simulink model "trim1031"  (R2023b)
settings: Solver=FixedStepAuto  StartTime=0.0  StopTime=200  FixedStep=0.01  RelTol=1e-3
model workspace (MAT data in the model file):
  op_trim1 = opcond.OperatingReport
  op_trim1.Outputs_ = opcond.OutputReport
  op_trim1.Outputs_.yspec_ = [0; 0; 0; 0; 0; 0; 0; 0; 0; 0; 0; 0]
  op_trim1.Outputs_.Block_ = 'trim1031/Output'
  op_trim1.Outputs_.PortWidth_ = 12
  op_trim1.Outputs_.PortNumber_ = NaN
  op_trim1.Outputs_.y_ = [0; 0.0983498986082; 0; -8.56242251282e-06; 0.0451960964113; 8.5624225128e-06; 119.999610613; 2.25043852977e-23; 15.9978397106; 0; 0; -1500.00000422]
  op_trim1.Outputs_.Known_ = [0; 0; 0; 0; 0; 0; 0; 0; 0; 0; 0; 0]
  op_trim1.Outputs_.Min_ = [-Inf; -Inf; -Inf; -Inf; -Inf; -Inf; -Inf; -Inf; -Inf; -Inf; -Inf; -Inf]
  op_trim1.Outputs_.Max_ = [Inf; Inf; Inf; Inf; Inf; Inf; Inf; Inf; Inf; Inf; Inf; Inf]
  op_trim1.TerminationString_ = '成功满足工作点设定。'
  op_trim1.OptimizationOutput_.iterations = 3
  op_trim1.OptimizationOutput_.funcCount = 44
  op_trim1.OptimizationOutput_.lssteplength = 1
  op_trim1.OptimizationOutput_.stepsize = 1.35481389825e-14
  op_trim1.OptimizationOutput_.algorithm = 'active-set'
  op_trim1.OptimizationOutput_.firstorderopt = 0
  op_trim1.OptimizationOutput_.constrviolation = 9.60120871696e-13
  op_trim1.OptimizationOutput_.message = '找到满足约束的局部最小值。
    | 
    | 优化已完成，因为目标函数沿
    | 可行方向在最优性容差值范围内呈现非递减，
    | 并且在约束容差值范围内满足约束。
    | 
    | <停止条件详细信息>
    | 
    | 优化已完成: 一阶最优性测度 0.000000e+00 小于
    | options.OptimalityTolerance = 1.000000e-06，并且最大约束违反值
    | 9.601209e-13 小于 options.ConstraintTolerance = 1.000000e-06。'
  op_trim1.OptimizationOutput_.bestfeasible.x = [0.0983498986082; -8.56242251282e-06; 0.0451960964113; 8.5624225128e-06; 119.999610613; 2.25043852977e-23; 15.9978397106; 0; -1500.00000422; -0.150930640428; 150000; 0; 0]
  op_trim1.OptimizationOutput_.bestfeasible.fval = 0
  op_trim1.OptimizationOutput_.bestfeasible.constrviolation = 9.60120871696e-13
  op_trim1.OptimizationOutput_.bestfeasible.firstorderopt = 0
  op_trim1.OptimizationOutput_.progress = {'<font face="monospaced"; size=3><BR>', '正在优化以求解所有所需的 dx/dt=0、x(k+1)-x(k)=0 和 y=ydes。<BR>', ' <BR>', '(最大误差)模块<BR>', ' ---------------------------------------------------------<BR>', '(4.86343e+00) trim1031/B747 Dynamics动力学参数计算/6DOF Equations of Motion运动学/6DOF (Euler Angles)1/Calculate DCM & Euler Angles/phi theta psi<BR>', '(3.43171e-05) trim1031/B747 Dynamics动力学参数计算/6DOF Equations of Motion运动学/6DOF (Euler Angles)1/Calculate DCM & Euler Angles/phi theta psi<BR>', '(9.60121e-13) trim1031/B747 Dynamics动力学参数计算/6DOF Equations of Motion运动学/6DOF (Euler Angles)1/Calculate DCM & Euler Angles/phi theta psi<BR>', '(9.60121e-13) trim1031/B747 Dynamics动力学参数计算/6DOF Equations of Motion运动学/6DOF (Euler Angles)1/Calculate DCM & Euler Angles/phi theta psi<BR>', ' <BR>', '成功满足工作点设定。<BR>'}
  op_trim1.Model_ = 'trim1031'
  op_trim1.States_(1) = opcond.StateReport
  op_trim1.States_(1).dx_ = [-7.71758340957e-06; 0.0451960964113; 8.60400095293e-06]
  op_trim1.States_(1).Nx_ = 3
  op_trim1.States_(1).Block_ = 'trim1031/B747 Dynamics动力学参数计算/6DOF Equations of Motion运动学/6DOF (Euler Angles)1/Calculate DCM &
    | Euler Angles/phi
    | theta
    | psi'
  op_trim1.States_(1).x_ = [0; 0.0983498986082; 0]
  op_trim1.States_(1).SteadyState_ = [0; 0; 0]
  op_trim1.States_(1).dxMin_ = [-0.3; -0.3; -0.3]
  op_trim1.States_(1).dxMax_ = [0.3; 0.3; 0.3]
  op_trim1.States_(1).Known_ = [1; 0; 1]
  op_trim1.States_(1).Min_ = [-0.5; -0.5; -0.5]
  op_trim1.States_(1).Max_ = [0.5; 0.5; 0.5]
  op_trim1.States_(2) = opcond.StateReport
  op_trim1.States_(2).dx_ = [9.49140044542e-06; 1.90507944892e-15; -1.25297191981e-06]
  op_trim1.States_(2).Nx_ = 3
  op_trim1.States_(2).Block_ = 'trim1031/B747 Dynamics动力学参数计算/6DOF Equations of Motion运动学/6DOF (Euler Angles)1/p,q,r '
  op_trim1.States_(2).x_ = [-8.56242251282e-06; 0.0451960964113; 8.5624225128e-06]
  op_trim1.States_(2).SteadyState_ = [0; 1; 0]
  op_trim1.States_(2).dxMin_ = [-Inf; -Inf; -Inf]
  op_trim1.States_(2).dxMax_ = [Inf; Inf; Inf]
  op_trim1.States_(2).Known_ = [0; 0; 0]
  op_trim1.States_(2).Min_ = [-0.3; -0.3; -0.3]
  op_trim1.States_(2).Max_ = [0.3; 0.3; 0.3]
  op_trim1.States_(3) = opcond.StateReport
  op_trim1.States_(3).dx_ = [0.251459835226; -0.00116446763034; -9.60120871696e-13]
  op_trim1.States_(3).Nx_ = 3
  op_trim1.States_(3).Block_ = 'trim1031/B747 Dynamics动力学参数计算/6DOF Equations of Motion运动学/6DOF (Euler Angles)1/ub,vb,wb'
  op_trim1.States_(3).x_ = [119.999610613; 2.25043852977e-23; 15.9978397106]
  op_trim1.States_(3).SteadyState_ = [0; 0; 1]
  op_trim1.States_(3).dxMin_ = [-Inf; -Inf; -Inf]
  op_trim1.States_(3).dxMax_ = [Inf; Inf; Inf]
  op_trim1.States_(3).Known_ = [0; 0; 0]
  op_trim1.States_(3).Min_ = [0; 0; 0]
  op_trim1.States_(3).Max_ = [Inf; Inf; Inf]
  op_trim1.States_(4) = opcond.StateReport
  op_trim1.States_(4).dx_ = [120.990568654; 2.25043852977e-23; 4.13759827182]
  op_trim1.States_(4).Nx_ = 3
  op_trim1.States_(4).Block_ = 'trim1031/B747 Dynamics动力学参数计算/6DOF Equations of Motion运动学/6DOF (Euler Angles)1/xe,ye,ze'
  op_trim1.States_(4).x_ = [0; 0; -1500.00000422]
  op_trim1.States_(4).SteadyState_ = [0; 1; 0]
  op_trim1.States_(4).dxMin_ = [-Inf; -Inf; -Inf]
  op_trim1.States_(4).dxMax_ = [Inf; Inf; Inf]
  op_trim1.States_(4).Known_ = [0; 1; 0]
  op_trim1.States_(4).Min_ = [-Inf; -Inf; -Inf]
  op_trim1.States_(4).Max_ = [Inf; Inf; 0]
  op_trim1.Inputs_(1) = opcond.InputReport
  op_trim1.Inputs_(1).Block_ = 'trim1031/dE'
  op_trim1.Inputs_(1).PortWidth_ = 1
  op_trim1.Inputs_(1).PortDimensions_ = [1 1]
  op_trim1.Inputs_(1).u_ = -0.150930640428
  op_trim1.Inputs_(1).Known_ = 0
  op_trim1.Inputs_(1).Min_ = -Inf
  op_trim1.Inputs_(1).Max_ = Inf
  op_trim1.Inputs_(2) = opcond.InputReport
  op_trim1.Inputs_(2).Block_ = 'trim1031/dT'
  op_trim1.Inputs_(2).PortWidth_ = 1
  op_trim1.Inputs_(2).PortDimensions_ = [1 1]
  op_trim1.Inputs_(2).u_ = 150000
  op_trim1.Inputs_(2).Known_ = 0
  op_trim1.Inputs_(2).Min_ = 0
  op_trim1.Inputs_(2).Max_ = 240000
  op_trim1.Inputs_(3) = opcond.InputReport
  op_trim1.Inputs_(3).Block_ = 'trim1031/dA'
  op_trim1.Inputs_(3).PortWidth_ = 1
  op_trim1.Inputs_(3).PortDimensions_ = [1 1]
  op_trim1.Inputs_(3).Known_ = 0
  op_trim1.Inputs_(3).Min_ = -Inf
  op_trim1.Inputs_(3).Max_ = Inf
  op_trim1.Inputs_(4) = opcond.InputReport
  op_trim1.Inputs_(4).Block_ = 'trim1031/dR'
  op_trim1.Inputs_(4).PortWidth_ = 1
  op_trim1.Inputs_(4).PortDimensions_ = [1 1]
  op_trim1.Inputs_(4).Known_ = 0
  op_trim1.Inputs_(4).Min_ = -Inf
  op_trim1.Inputs_(4).Max_ = Inf
  op_trim10 = opcond.OperatingReport
  op_trim10.Outputs_ = opcond.OutputReport
  op_trim10.Outputs_.yspec_ = [0; 0; 0; 0; 0; 0; 0; 0; 0; 0; 0; 0]
  op_trim10.Outputs_.Block_ = 'trim1031/Output'
  op_trim10.Outputs_.PortWidth_ = 12
  op_trim10.Outputs_.PortNumber_ = NaN
  op_trim10.Outputs_.y_ = [0; 0.171651347214; 0; -1.07398465823e-08; -0.0379829933296; 1.07398466044e-08; 130.000005709; 9.36786863606e-26; 0.00125401201938; 0; 0; -1499.99999996]
  op_trim10.Outputs_.Known_ = [0; 0; 0; 0; 0; 0; 0; 0; 0; 0; 0; 0]
  op_trim10.Outputs_.Min_ = [-Inf; -Inf; -Inf; -Inf; -Inf; -Inf; -Inf; -Inf; -Inf; -Inf; -Inf; -Inf]
  op_trim10.Outputs_.Max_ = [Inf; Inf; Inf; Inf; Inf; Inf; Inf; Inf; Inf; Inf; Inf; Inf]
  op_trim10.TerminationString_ = '成功满足工作点设定。'
  op_trim10.OptimizationOutput_.iterations = 3
  op_trim10.OptimizationOutput_.funcCount = 44
  op_trim10.OptimizationOutput_.lssteplength = 1
  op_trim10.OptimizationOutput_.stepsize = 3.37664542003e-16
  op_trim10.OptimizationOutput_.algorithm = 'active-set'
  op_trim10.OptimizationOutput_.firstorderopt = 0
  op_trim10.OptimizationOutput_.constrviolation = 2.30926389122e-14
  op_trim10.OptimizationOutput_.message = '找到满足约束的局部最小值。
    | 
    | 优化已完成，因为目标函数沿
    | 可行方向在最优性容差值范围内呈现非递减，
    | 并且在约束容差值范围内满足约束。
    | 
    | <停止条件详细信息>
    | 
    | 优化已完成: 一阶最优性测度 0.000000e+00 小于
    | options.OptimalityTolerance = 1.000000e-06，并且最大约束违反值
    | 2.309264e-14 小于 options.ConstraintTolerance = 1.000000e-06。'
  op_trim10.OptimizationOutput_.bestfeasible.x = [0.171651347214; -1.07398465823e-08; -0.0379829933296; 1.07398466044e-08; 130.000005709; 9.36786863606e-26; 0.00125401201938; 0; -1499.99999996; 0.0383261837012; 192000; 0; 0]
  op_trim10.OptimizationOutput_.bestfeasible.fval = 0
  op_trim10.OptimizationOutput_.bestfeasible.constrviolation = 2.30926389122e-14
  op_trim10.OptimizationOutput_.bestfeasible.firstorderopt = 0
  op_trim10.OptimizationOutput_.progress = {'<font face="monospaced"; size=3><BR>', '正在优化以求解所有所需的 dx/dt=0、x(k+1)-x(k)=0 和 y=ydes。<BR>', ' <BR>', '(最大误差)模块<BR>', ' ---------------------------------------------------------<BR>', '(5.22143e+00) trim1031/B747 Dynamics动力学参数计算/6DOF Equations of Motion运动学/6DOF (Euler Angles)1/p,q,r <BR>', '(1.34354e-05) trim1031/B747 Dynamics动力学参数计算/6DOF Equations of Motion运动学/6DOF (Euler Angles)1/p,q,r <BR>', '(2.30926e-14) trim1031/B747 Dynamics动力学参数计算/6DOF Equations of Motion运动学/6DOF (Euler Angles)1/p,q,r <BR>', '(2.30926e-14) trim1031/B747 Dynamics动力学参数计算/6DOF Equations of Motion运动学/6DOF (Euler Angles)1/p,q,r <BR>', ' <BR>', '成功满足工作点设定。<BR>'}
  op_trim10.Model_ = 'trim1031'
  op_trim10.States_(1) = opcond.StateReport
  op_trim10.States_(1).dx_ = [-8.87801564728e-09; -0.0379829933296; 1.09000330053e-08]
  op_trim10.States_(1).Nx_ = 3
  op_trim10.States_(1).Block_ = 'trim1031/B747 Dynamics动力学参数计算/6DOF Equations of Motion运动学/6DOF (Euler Angles)1/Calculate DCM &
    | Euler Angles/phi
    | theta
    | psi'
  op_trim10.States_(1).x_ = [0; 0.171651347214; 0]
  op_trim10.States_(1).SteadyState_ = [0; 0; 0]
  op_trim10.States_(1).dxMin_ = [-0.3; -0.3; -0.3]
  op_trim10.States_(1).dxMax_ = [0.3; 0.3; 0.3]
  op_trim10.States_(1).Known_ = [1; 0; 1]
  op_trim10.States_(1).Min_ = [-0.5; -0.5; -0.5]
  op_trim10.States_(1).Max_ = [0.5; 0.5; 0.5]
  op_trim10.States_(2) = opcond.StateReport
  op_trim10.States_(2).dx_ = [1.28499584643e-08; -1.21202080755e-16; -2.5916435012e-09]
  op_trim10.States_(2).Nx_ = 3
  op_trim10.States_(2).Block_ = 'trim1031/B747 Dynamics动力学参数计算/6DOF Equations of Motion运动学/6DOF (Euler Angles)1/p,q,r '
  op_trim10.States_(2).x_ = [-1.07398465823e-08; -0.0379829933296; 1.07398466044e-08]
  op_trim10.States_(2).SteadyState_ = [0; 1; 0]
  op_trim10.States_(2).dxMin_ = [-0.03; -0.03; -0.03]
  op_trim10.States_(2).dxMax_ = [0.03; 0.03; 0.03]
  op_trim10.States_(2).Known_ = [0; 0; 0]
  op_trim10.States_(2).Min_ = [-0.3; -0.3; -0.3]
  op_trim10.States_(2).Max_ = [0.3; 0.3; 0.3]
  op_trim10.States_(3) = opcond.StateReport
  op_trim10.States_(3).dx_ = [-1.06099582482; -1.39619358779e-06; -2.30926389122e-14]
  op_trim10.States_(3).Nx_ = 3
  op_trim10.States_(3).Block_ = 'trim1031/B747 Dynamics动力学参数计算/6DOF Equations of Motion运动学/6DOF (Euler Angles)1/ub,vb,wb'
  op_trim10.States_(3).x_ = [130.000005709; 9.36786863606e-26; 0.00125401201938]
  op_trim10.States_(3).SteadyState_ = [0; 0; 1]
  op_trim10.States_(3).dxMin_ = [-Inf; -Inf; -Inf]
  op_trim10.States_(3).dxMax_ = [Inf; Inf; Inf]
  op_trim10.States_(3).Known_ = [0; 0; 0]
  op_trim10.States_(3).Min_ = [0; 0; 0]
  op_trim10.States_(3).Max_ = [Inf; Inf; Inf]
  op_trim10.States_(4) = opcond.StateReport
  op_trim10.States_(4).dx_ = [128.089745597; 9.36786863606e-26; -22.2040212324]
  op_trim10.States_(4).Nx_ = 3
  op_trim10.States_(4).Block_ = 'trim1031/B747 Dynamics动力学参数计算/6DOF Equations of Motion运动学/6DOF (Euler Angles)1/xe,ye,ze'
  op_trim10.States_(4).x_ = [0; 0; -1499.99999996]
  op_trim10.States_(4).SteadyState_ = [0; 1; 0]
  op_trim10.States_(4).dxMin_ = [-Inf; -Inf; -Inf]
  op_trim10.States_(4).dxMax_ = [Inf; Inf; Inf]
  op_trim10.States_(4).Known_ = [0; 1; 0]
  op_trim10.States_(4).Min_ = [-Inf; -Inf; -Inf]
  op_trim10.States_(4).Max_ = [Inf; Inf; 0]
  op_trim10.Inputs_(1) = opcond.InputReport
  op_trim10.Inputs_(1).Block_ = 'trim1031/dE'
  op_trim10.Inputs_(1).PortWidth_ = 1
  op_trim10.Inputs_(1).PortDimensions_ = [1 1]
  op_trim10.Inputs_(1).u_ = 0.0383261837012
  op_trim10.Inputs_(1).Known_ = 0
  op_trim10.Inputs_(1).Min_ = -Inf
  op_trim10.Inputs_(1).Max_ = Inf
  op_trim10.Inputs_(2) = opcond.InputReport
  op_trim10.Inputs_(2).Block_ = 'trim1031/dT'
  op_trim10.Inputs_(2).PortWidth_ = 1
  op_trim10.Inputs_(2).PortDimensions_ = [1 1]
  op_trim10.Inputs_(2).u_ = 192000
  op_trim10.Inputs_(2).Known_ = 0
  op_trim10.Inputs_(2).Min_ = 0
  op_trim10.Inputs_(2).Max_ = 240000
  op_trim10.Inputs_(3) = opcond.InputReport
  op_trim10.Inputs_(3).Block_ = 'trim1031/dA'
  op_trim10.Inputs_(3).PortWidth_ = 1
  op_trim10.Inputs_(3).PortDimensions_ = [1 1]
  op_trim10.Inputs_(3).Known_ = 0
  op_trim10.Inputs_(3).Min_ = -Inf
  op_trim10.Inputs_(3).Max_ = Inf
  op_trim10.Inputs_(4) = opcond.InputReport
  op_trim10.Inputs_(4).Block_ = 'trim1031/dR'
  op_trim10.Inputs_(4).PortWidth_ = 1
  op_trim10.Inputs_(4).PortDimensions_ = [1 1]
  op_trim10.Inputs_(4).Known_ = 0
  op_trim10.Inputs_(4).Min_ = -Inf
  op_trim10.Inputs_(4).Max_ = Inf
  op_trim11 = opcond.OperatingReport
  op_trim11.Outputs_ = opcond.OutputReport
  op_trim11.Outputs_.yspec_ = [0; 0; 0; 0; 0; 0; 0; 0; 0; 0; 0; 0]
  op_trim11.Outputs_.Block_ = 'trim1031/Output'
  op_trim11.Outputs_.PortWidth_ = 12
  op_trim11.Outputs_.PortNumber_ = NaN
  op_trim11.Outputs_.y_ = [0; 0.168996963218; 0; -9.68112442029e-09; 0.0390344222981; 9.6811244158e-09; 129.999918266; 0; 12.9993206248; 0; 0; -1500.0000011]
  op_trim11.Outputs_.Known_ = [0; 0; 0; 0; 0; 0; 0; 0; 0; 0; 0; 0]
  op_trim11.Outputs_.Min_ = [-Inf; -Inf; -Inf; -Inf; -Inf; -Inf; -Inf; -Inf; -Inf; -Inf; -Inf; -Inf]
  op_trim11.Outputs_.Max_ = [Inf; Inf; Inf; Inf; Inf; Inf; Inf; Inf; Inf; Inf; Inf; Inf]
  op_trim11.TerminationString_ = '成功满足工作点设定。'
  op_trim11.OptimizationOutput_.iterations = 4
  op_trim11.OptimizationOutput_.funcCount = 59
  op_trim11.OptimizationOutput_.lssteplength = 1
  op_trim11.OptimizationOutput_.stepsize = 2.96700940297e-15
  op_trim11.OptimizationOutput_.algorithm = 'active-set'
  op_trim11.OptimizationOutput_.firstorderopt = 0
  op_trim11.OptimizationOutput_.constrviolation = 1.7763568394e-14
  op_trim11.OptimizationOutput_.message = '找到满足约束的局部最小值。
    | 
    | 优化已完成，因为目标函数沿
    | 可行方向在最优性容差值范围内呈现非递减，
    | 并且在约束容差值范围内满足约束。
    | 
    | <停止条件详细信息>
    | 
    | 优化已完成: 一阶最优性测度 0.000000e+00 小于
    | options.OptimalityTolerance = 1.000000e-06，并且最大约束违反值
    | 1.776357e-14 小于 options.ConstraintTolerance = 1.000000e-06。'
  op_trim11.OptimizationOutput_.bestfeasible.x = [0.168996963218; -9.68112442029e-09; 0.0390344222981; 9.6811244158e-09; 129.999918266; 0; 12.9993206248; 0; -1500.0000011; -0.0881300190709; 192000; 0; 0]
  op_trim11.OptimizationOutput_.bestfeasible.fval = 0
  op_trim11.OptimizationOutput_.bestfeasible.constrviolation = 1.7763568394e-14
  op_trim11.OptimizationOutput_.bestfeasible.firstorderopt = 0
  op_trim11.OptimizationOutput_.progress = {'<font face="monospaced"; size=3><BR>', '正在优化以求解所有所需的 dx/dt=0、x(k+1)-x(k)=0 和 y=ydes。<BR>', ' <BR>', '(最大误差)模块<BR>', ' ---------------------------------------------------------<BR>', '(4.97990e+00) trim1031/B747 Dynamics动力学参数计算/6DOF Equations of Motion运动学/6DOF (Euler Angles)1/p,q,r <BR>', '(4.08961e-02) trim1031/B747 Dynamics动力学参数计算/6DOF Equations of Motion运动学/6DOF (Euler Angles)1/Calculate DCM & Euler Angles/phi theta psi<BR>', '(1.05395e-06) trim1031/B747 Dynamics动力学参数计算/6DOF Equations of Motion运动学/6DOF (Euler Angles)1/p,q,r <BR>', '(1.77636e-14) trim1031/B747 Dynamics动力学参数计算/6DOF Equations of Motion运动学/6DOF (Euler Angles)1/p,q,r <BR>', '(1.77636e-14) trim1031/B747 Dynamics动力学参数计算/6DOF Equations of Motion运动学/6DOF (Euler Angles)1/p,q,r <BR>', ' <BR>', '成功满足工作点设定。<BR>'}
  op_trim11.Model_ = 'trim1031'
  op_trim11.States_(1) = opcond.StateReport
  op_trim11.States_(1).dx_ = [-8.02928830529e-09; 0.0390344222981; 9.82103520536e-09]
  op_trim11.States_(1).Nx_ = 3
  op_trim11.States_(1).Block_ = 'trim1031/B747 Dynamics动力学参数计算/6DOF Equations of Motion运动学/6DOF (Euler Angles)1/Calculate DCM &
    | Euler Angles/phi
    | theta
    | psi'
  op_trim11.States_(1).x_ = [0; 0.168996963218; 0]
  op_trim11.States_(1).SteadyState_ = [0; 0; 0]
  op_trim11.States_(1).dxMin_ = [-0.3; -0.3; -0.3]
  op_trim11.States_(1).dxMax_ = [0.3; 0.3; 0.3]
  op_trim11.States_(1).Known_ = [1; 0; 1]
  op_trim11.States_(1).Min_ = [-0.5; -0.5; -0.5]
  op_trim11.States_(1).Max_ = [0.5; 0.5; 0.5]
  op_trim11.States_(2) = opcond.StateReport
  op_trim11.States_(2).dx_ = [1.15109176436e-08; -0.03; -1.70079708465e-09]
  op_trim11.States_(2).Nx_ = 3
  op_trim11.States_(2).Block_ = 'trim1031/B747 Dynamics动力学参数计算/6DOF Equations of Motion运动学/6DOF (Euler Angles)1/p,q,r '
  op_trim11.States_(2).x_ = [-9.68112442029e-09; 0.0390344222981; 9.6811244158e-09]
  op_trim11.States_(2).SteadyState_ = [0; 0; 0]
  op_trim11.States_(2).dxMin_ = [-0.03; -0.03; -0.03]
  op_trim11.States_(2).dxMax_ = [0.03; 0.03; 0.03]
  op_trim11.States_(2).Known_ = [0; 0; 0]
  op_trim11.States_(2).Min_ = [-0.3; -0.3; -0.3]
  op_trim11.States_(2).Max_ = [0.3; 0.3; 0.3]
  op_trim11.States_(3) = opcond.StateReport
  op_trim11.States_(3).dx_ = [-0.537845537105; -1.38439342313e-06; -1.7763568394e-14]
  op_trim11.States_(3).Nx_ = 3
  op_trim11.States_(3).Block_ = 'trim1031/B747 Dynamics动力学参数计算/6DOF Equations of Motion运动学/6DOF (Euler Angles)1/ub,vb,wb'
  op_trim11.States_(3).x_ = [129.999918266; 0; 12.9993206248]
  op_trim11.States_(3).SteadyState_ = [0; 0; 1]
  op_trim11.States_(3).dxMin_ = [-Inf; -Inf; -Inf]
  op_trim11.States_(3).dxMax_ = [Inf; Inf; Inf]
  op_trim11.States_(3).Known_ = [0; 0; 0]
  op_trim11.States_(3).Min_ = [0; 0; 0]
  op_trim11.States_(3).Max_ = [Inf; Inf; Inf]
  op_trim11.States_(4) = opcond.StateReport
  op_trim11.States_(4).dx_ = [130.334338824; 0; -9.05103360207]
  op_trim11.States_(4).Nx_ = 3
  op_trim11.States_(4).Block_ = 'trim1031/B747 Dynamics动力学参数计算/6DOF Equations of Motion运动学/6DOF (Euler Angles)1/xe,ye,ze'
  op_trim11.States_(4).x_ = [0; 0; -1500.0000011]
  op_trim11.States_(4).SteadyState_ = [0; 1; 0]
  op_trim11.States_(4).dxMin_ = [-Inf; -Inf; -Inf]
  op_trim11.States_(4).dxMax_ = [Inf; Inf; Inf]
  op_trim11.States_(4).Known_ = [0; 1; 0]
  op_trim11.States_(4).Min_ = [-Inf; -Inf; -Inf]
  op_trim11.States_(4).Max_ = [Inf; Inf; 0]
  op_trim11.Inputs_(1) = opcond.InputReport
  op_trim11.Inputs_(1).Block_ = 'trim1031/dE'
  op_trim11.Inputs_(1).PortWidth_ = 1
  op_trim11.Inputs_(1).PortDimensions_ = [1 1]
  op_trim11.Inputs_(1).u_ = -0.0881300190709
  op_trim11.Inputs_(1).Known_ = 0
  op_trim11.Inputs_(1).Min_ = -Inf
  op_trim11.Inputs_(1).Max_ = Inf
  op_trim11.Inputs_(2) = opcond.InputReport
  op_trim11.Inputs_(2).Block_ = 'trim1031/dT'
  op_trim11.Inputs_(2).PortWidth_ = 1
  op_trim11.Inputs_(2).PortDimensions_ = [1 1]
  op_trim11.Inputs_(2).u_ = 192000
  op_trim11.Inputs_(2).Known_ = 0
  op_trim11.Inputs_(2).Min_ = 0
  op_trim11.Inputs_(2).Max_ = 240000
  op_trim11.Inputs_(3) = opcond.InputReport
  op_trim11.Inputs_(3).Block_ = 'trim1031/dA'
  op_trim11.Inputs_(3).PortWidth_ = 1
  op_trim11.Inputs_(3).PortDimensions_ = [1 1]
  op_trim11.Inputs_(3).Known_ = 0
  op_trim11.Inputs_(3).Min_ = -Inf
  op_trim11.Inputs_(3).Max_ = Inf
  op_trim11.Inputs_(4) = opcond.InputReport
  op_trim11.Inputs_(4).Block_ = 'trim1031/dR'
  op_trim11.Inputs_(4).PortWidth_ = 1
  op_trim11.Inputs_(4).PortDimensions_ = [1 1]
  op_trim11.Inputs_(4).Known_ = 0
  op_trim11.Inputs_(4).Min_ = -Inf
  op_trim11.Inputs_(4).Max_ = Inf
  op_trim12 = opcond.OperatingReport
  op_trim12.Outputs_ = opcond.OutputReport
  op_trim12.Outputs_.yspec_ = [0; 0; 0; 0; 0; 0; 0; 0; 0; 0; 0; 0]
  op_trim12.Outputs_.Block_ = 'trim1031/Output'
  op_trim12.Outputs_.PortWidth_ = 12
  op_trim12.Outputs_.PortNumber_ = NaN
  op_trim12.Outputs_.y_ = [0; 0.167988525312; 0; 1.78845872578e-25; -0.00250420987712; 1e-05; 129.999998768; -2.5381879176e-33; 13.0000321666; 0; 0; -1499.99999999]
  op_trim12.Outputs_.Known_ = [0; 0; 0; 0; 0; 0; 0; 0; 0; 0; 0; 0]
  op_trim12.Outputs_.Min_ = [-Inf; -Inf; -Inf; -Inf; -Inf; -Inf; -Inf; -Inf; -Inf; -Inf; -Inf; -Inf]
  op_trim12.Outputs_.Max_ = [Inf; Inf; Inf; Inf; Inf; Inf; Inf; Inf; Inf; Inf; Inf; Inf]
  op_trim12.TerminationString_ = '成功满足工作点设定。'
  op_trim12.OptimizationOutput_.iterations = 2
  op_trim12.OptimizationOutput_.funcCount = 44
  op_trim12.OptimizationOutput_.lssteplength = 1
  op_trim12.OptimizationOutput_.stepsize = 2.2121751606e-07
  op_trim12.OptimizationOutput_.algorithm = 'active-set'
  op_trim12.OptimizationOutput_.firstorderopt = 2.36442055551e-11
  op_trim12.OptimizationOutput_.constrviolation = 1.41622824579e-14
  op_trim12.OptimizationOutput_.message = '找到满足约束的局部最小值。
    | 
    | 优化已完成，因为目标函数沿
    | 可行方向在最优性容差值范围内呈现非递减，
    | 并且在约束容差值范围内满足约束。
    | 
    | <停止条件详细信息>
    | 
    | 优化已完成: 一阶最优性测度 2.364421e-11 小于
    | options.OptimalityTolerance = 1.000000e-06，并且最大约束违反值
    | 1.416228e-14 小于 options.ConstraintTolerance = 1.000000e-06。'
  op_trim12.OptimizationOutput_.bestfeasible.x = [0.167988525312; 1.78845872578e-25; -0.00250420987712; 1e-05; 129.999998768; -2.5381879176e-33; 13.0000321666; 0; -1499.99999999; -0.0498466910775; 192000; 0; 0]
  op_trim12.OptimizationOutput_.bestfeasible.fval = 0
  op_trim12.OptimizationOutput_.bestfeasible.constrviolation = 1.41622824579e-14
  op_trim12.OptimizationOutput_.bestfeasible.firstorderopt = 2.36442055551e-11
  op_trim12.OptimizationOutput_.progress = {'<font face="monospaced"; size=3><BR>', '正在优化以求解所有所需的 dx/dt=0、x(k+1)-x(k)=0 和 y=ydes。<BR>', ' <BR>', '(最大误差)模块<BR>', ' ---------------------------------------------------------<BR>', '(4.96933e-02) trim1031/B747 Dynamics动力学参数计算/6DOF Equations of Motion运动学/6DOF (Euler Angles)1/p,q,r <BR>', '(3.41872e-06) trim1031/B747 Dynamics动力学参数计算/6DOF Equations of Motion运动学/6DOF (Euler Angles)1/p,q,r <BR>', '(1.41623e-14) trim1031/B747 Dynamics动力学参数计算/6DOF Equations of Motion运动学/6DOF (Euler Angles)1/p,q,r <BR>', '(1.41623e-14) trim1031/B747 Dynamics动力学参数计算/6DOF Equations of Motion运动学/6DOF (Euler Angles)1/p,q,r <BR>', ' <BR>', '成功满足工作点设定。<BR>'}
  op_trim12.Model_ = 'trim1031'
  op_trim12.States_(1) = opcond.StateReport
  op_trim12.States_(1).dx_ = [1.69586789196e-06; -0.00250420987712; 1.01427791018e-05]
  op_trim12.States_(1).Nx_ = 3
  op_trim12.States_(1).Block_ = 'trim1031/B747 Dynamics动力学参数计算/6DOF Equations of Motion运动学/6DOF (Euler Angles)1/Calculate DCM &
    | Euler Angles/phi
    | theta
    | psi'
  op_trim12.States_(1).x_ = [0; 0.167988525312; 0]
  op_trim12.States_(1).SteadyState_ = [0; 0; 0]
  op_trim12.States_(1).dxMin_ = [-0.3; -0.3; -0.3]
  op_trim12.States_(1).dxMax_ = [0.3; 0.3; 0.3]
  op_trim12.States_(1).Known_ = [1; 0; 1]
  op_trim12.States_(1).Min_ = [-0.5; -0.5; -0.5]
  op_trim12.States_(1).Max_ = [0.5; 0.5; 0.5]
  op_trim12.States_(2) = opcond.StateReport
  op_trim12.States_(2).dx_ = [3.92855222752e-06; -0.0262934164576; -2.41695804279e-06]
  op_trim12.States_(2).Nx_ = 3
  op_trim12.States_(2).Block_ = 'trim1031/B747 Dynamics动力学参数计算/6DOF Equations of Motion运动学/6DOF (Euler Angles)1/p,q,r '
  op_trim12.States_(2).x_ = [1.78845872578e-25; -0.00250420987712; 1e-05]
  op_trim12.States_(2).SteadyState_ = [0; 0; 0]
  op_trim12.States_(2).dxMin_ = [-0.03; -0.03; -0.03]
  op_trim12.States_(2).dxMax_ = [0.03; 0.03; 0.03]
  op_trim12.States_(2).Known_ = [0; 0; 0]
  op_trim12.States_(2).Min_ = [-0.3; -0.3; -0.3]
  op_trim12.States_(2).Max_ = [0.3; 0.3; 0.3]
  op_trim12.States_(3) = opcond.StateReport
  op_trim12.States_(3).dx_ = [1.41622824579e-14; -0.00129999998768; -5.27904040513]
  op_trim12.States_(3).Nx_ = 3
  op_trim12.States_(3).Block_ = 'trim1031/B747 Dynamics动力学参数计算/6DOF Equations of Motion运动学/6DOF (Euler Angles)1/ub,vb,wb'
  op_trim12.States_(3).x_ = [129.999998768; -2.5381879176e-33; 13.0000321666]
  op_trim12.States_(3).SteadyState_ = [1; 0; 0]
  op_trim12.States_(3).dxMin_ = [-Inf; -Inf; -Inf]
  op_trim12.States_(3).dxMax_ = [Inf; Inf; Inf]
  op_trim12.States_(3).Known_ = [0; 0; 0]
  op_trim12.States_(3).Min_ = [0; 0; 0]
  op_trim12.States_(3).Max_ = [Inf; Inf; Inf]
  op_trim12.States_(4) = opcond.StateReport
  op_trim12.States_(4).dx_ = [130.343598294; -2.5381879176e-33; -8.9189068687]
  op_trim12.States_(4).Nx_ = 3
  op_trim12.States_(4).Block_ = 'trim1031/B747 Dynamics动力学参数计算/6DOF Equations of Motion运动学/6DOF (Euler Angles)1/xe,ye,ze'
  op_trim12.States_(4).x_ = [0; 0; -1499.99999999]
  op_trim12.States_(4).SteadyState_ = [0; 1; 0]
  op_trim12.States_(4).dxMin_ = [-Inf; -Inf; -Inf]
  op_trim12.States_(4).dxMax_ = [Inf; Inf; Inf]
  op_trim12.States_(4).Known_ = [0; 1; 0]
  op_trim12.States_(4).Min_ = [-Inf; -Inf; -Inf]
  op_trim12.States_(4).Max_ = [Inf; Inf; 0]
  op_trim12.Inputs_(1) = opcond.InputReport
  op_trim12.Inputs_(1).Block_ = 'trim1031/dE'
  op_trim12.Inputs_(1).PortWidth_ = 1
  op_trim12.Inputs_(1).PortDimensions_ = [1 1]
  op_trim12.Inputs_(1).u_ = -0.0498466910775
  op_trim12.Inputs_(1).Known_ = 0
  op_trim12.Inputs_(1).Min_ = -Inf
  op_trim12.Inputs_(1).Max_ = Inf
  op_trim12.Inputs_(2) = opcond.InputReport
  op_trim12.Inputs_(2).Block_ = 'trim1031/dT'
  op_trim12.Inputs_(2).PortWidth_ = 1
  op_trim12.Inputs_(2).PortDimensions_ = [1 1]
  op_trim12.Inputs_(2).u_ = 192000
  op_trim12.Inputs_(2).Known_ = 0
  op_trim12.Inputs_(2).Min_ = 0
  op_trim12.Inputs_(2).Max_ = 240000
  op_trim12.Inputs_(3) = opcond.InputReport
  op_trim12.Inputs_(3).Block_ = 'trim1031/dA'
  op_trim12.Inputs_(3).PortWidth_ = 1
  op_trim12.Inputs_(3).PortDimensions_ = [1 1]
  op_trim12.Inputs_(3).Known_ = 0
  op_trim12.Inputs_(3).Min_ = -Inf
  op_trim12.Inputs_(3).Max_ = Inf
  op_trim12.Inputs_(4) = opcond.InputReport
  op_trim12.Inputs_(4).Block_ = 'trim1031/dR'
  op_trim12.Inputs_(4).PortWidth_ = 1
  op_trim12.Inputs_(4).PortDimensions_ = [1 1]
  op_trim12.Inputs_(4).Known_ = 0
  op_trim12.Inputs_(4).Min_ = -Inf
  op_trim12.Inputs_(4).Max_ = Inf
  op_trim13 = opcond.OperatingReport
  op_trim13.Outputs_ = opcond.OutputReport
  op_trim13.Outputs_.yspec_ = [0; 0; 0; 0; 0; 0; 0; 0; 0; 0; 0; 0]
  op_trim13.Outputs_.Block_ = 'trim1031/Output'
  op_trim13.Outputs_.PortWidth_ = 12
  op_trim13.Outputs_.PortNumber_ = NaN
  op_trim13.Outputs_.y_ = [0.0001; 0.1; 6.28308530718; -0.000179538158685; -0.00751789694975; -1.41195963211e-05; 121.02593479; 0.0127716364451; 6.63287181793; -2.82407339315e-17; 0; -1499.99553412]
  op_trim13.Outputs_.Known_ = [0; 0; 0; 0; 0; 0; 0; 0; 0; 0; 0; 0]
  op_trim13.Outputs_.Min_ = [-Inf; -Inf; -Inf; -Inf; -Inf; -Inf; -Inf; -Inf; -Inf; -Inf; -Inf; -Inf]
  op_trim13.Outputs_.Max_ = [Inf; Inf; Inf; Inf; Inf; Inf; Inf; Inf; Inf; Inf; Inf; Inf]
  op_trim13.TerminationString_ = '成功满足工作点设定。'
  op_trim13.OptimizationOutput_.iterations = 4
  op_trim13.OptimizationOutput_.funcCount = 55
  op_trim13.OptimizationOutput_.lssteplength = 1
  op_trim13.OptimizationOutput_.stepsize = 1.07319719222e-09
  op_trim13.OptimizationOutput_.algorithm = 'active-set'
  op_trim13.OptimizationOutput_.firstorderopt = 0
  op_trim13.OptimizationOutput_.constrviolation = 2.33658647986e-11
  op_trim13.OptimizationOutput_.message = '找到满足约束的局部最小值。
    | 
    | 优化已完成，因为目标函数沿
    | 可行方向在最优性容差值范围内呈现非递减，
    | 并且在约束容差值范围内满足约束。
    | 
    | <停止条件详细信息>
    | 
    | 优化已完成: 一阶最优性测度 0.000000e+00 小于
    | options.OptimalityTolerance = 1.000000e-06，并且最大约束违反值
    | 2.336586e-11 小于 options.ConstraintTolerance = 1.000000e-06。'
  op_trim13.OptimizationOutput_.bestfeasible.x = [-0.000179538158685; -0.00751789694975; -1.41195963211e-05; 121.02593479; 0.0127716364451; 6.63287181793; -2.82407339315e-17; -1499.99553412; -0.0124968353108; 191999.999642; -2.78444784735e-05; 0.00018916555193]
  op_trim13.OptimizationOutput_.bestfeasible.fval = 0
  op_trim13.OptimizationOutput_.bestfeasible.constrviolation = 2.33658647986e-11
  op_trim13.OptimizationOutput_.bestfeasible.firstorderopt = 0
  op_trim13.OptimizationOutput_.progress = {'<font face="monospaced"; size=3><BR>', '正在优化以求解所有所需的 dx/dt=0、x(k+1)-x(k)=0 和 y=ydes。<BR>', ' <BR>', '(最大误差)模块<BR>', ' ---------------------------------------------------------<BR>', '(1.84926e-01) trim1031/B747 Dynamics动力学参数计算/6DOF Equations of Motion运动学/6DOF (Euler Angles)1/xe,ye,ze<BR>', '(6.48574e-03) trim1031/B747 Dynamics动力学参数计算/6DOF Equations of Motion运动学/6DOF (Euler Angles)1/xe,ye,ze<BR>', '(9.24667e-06) trim1031/B747 Dynamics动力学参数计算/6DOF Equations of Motion运动学/6DOF (Euler Angles)1/xe,ye,ze<BR>', '(2.33659e-11) trim1031/B747 Dynamics动力学参数计算/6DOF Equations of Motion运动学/6DOF (Euler Angles)1/p,q,r <BR>', '(2.33659e-11) trim1031/B747 Dynamics动力学参数计算/6DOF Equations of Motion运动学/6DOF (Euler Angles)1/p,q,r <BR>', ' <BR>', '成功满足工作点设定。<BR>'}
  op_trim13.Model_ = 'trim1031'
  op_trim13.States_(1) = opcond.StateReport
  op_trim13.States_(1).dx_ = [-0.000181030274317; -0.0075178955002; -1.49460539596e-05]
  op_trim13.States_(1).Nx_ = 3
  op_trim13.States_(1).Block_ = 'trim1031/B747 Dynamics动力学参数计算/6DOF Equations of Motion运动学/6DOF (Euler Angles)1/Calculate DCM &
    | Euler Angles/phi
    | theta
    | psi'
  op_trim13.States_(1).x_ = [0.0001; 0.1; -0.0001]
  op_trim13.States_(1).SteadyState_ = [0; 0; 0]
  op_trim13.States_(1).dxMin_ = [-Inf; -0.2; -Inf]
  op_trim13.States_(1).dxMax_ = [Inf; 0.2; Inf]
  op_trim13.States_(1).Known_ = [1; 1; 1]
  op_trim13.States_(1).Min_ = [-Inf; -0.51; -Inf]
  op_trim13.States_(1).Max_ = [Inf; 0.51; Inf]
  op_trim13.States_(2) = opcond.StateReport
  op_trim13.States_(2).dx_ = [-3.34973655326e-15; -0.0200000000005; 5.67519754943e-15]
  op_trim13.States_(2).Nx_ = 3
  op_trim13.States_(2).Block_ = 'trim1031/B747 Dynamics动力学参数计算/6DOF Equations of Motion运动学/6DOF (Euler Angles)1/p,q,r '
  op_trim13.States_(2).x_ = [-0.000179538158685; -0.00751789694975; -1.41195963211e-05]
  op_trim13.States_(2).SteadyState_ = [1; 0; 1]
  op_trim13.States_(2).dxMin_ = [-Inf; -0.02; -Inf]
  op_trim13.States_(2).dxMax_ = [Inf; 0.02; Inf]
  op_trim13.States_(2).Known_ = [0; 0; 0]
  op_trim13.States_(2).Min_ = [-Inf; -0.2; -Inf]
  op_trim13.States_(2).Max_ = [Inf; 0.2; Inf]
  op_trim13.States_(3) = opcond.StateReport
  op_trim13.States_(3).dx_ = [1.83950285559e-11; -1.552358719e-12; -2.33658647986e-11]
  op_trim13.States_(3).Nx_ = 3
  op_trim13.States_(3).Block_ = 'trim1031/B747 Dynamics动力学参数计算/6DOF Equations of Motion运动学/6DOF (Euler Angles)1/ub,vb,wb'
  op_trim13.States_(3).x_ = [121.02593479; 0.0127716364451; 6.63287181793]
  op_trim13.States_(3).SteadyState_ = [1; 1; 1]
  op_trim13.States_(3).dxMin_ = [-Inf; -Inf; -Inf]
  op_trim13.States_(3).dxMax_ = [Inf; Inf; Inf]
  op_trim13.States_(3).Known_ = [0; 0; 0]
  op_trim13.States_(3).Min_ = [0; 0; 0]
  op_trim13.States_(3).Max_ = [Inf; Inf; Inf]
  op_trim13.States_(4) = opcond.StateReport
  op_trim13.States_(4).dx_ = [121.083492208; 1.99493199737e-17; -5.48269624853]
  op_trim13.States_(4).Nx_ = 3
  op_trim13.States_(4).Block_ = 'trim1031/B747 Dynamics动力学参数计算/6DOF Equations of Motion运动学/6DOF (Euler Angles)1/xe,ye,ze'
  op_trim13.States_(4).x_ = [-2.82407339315e-17; 0; -1499.99553412]
  op_trim13.States_(4).SteadyState_ = [0; 1; 0]
  op_trim13.States_(4).dxMin_ = [-Inf; -Inf; -100]
  op_trim13.States_(4).dxMax_ = [Inf; Inf; 100]
  op_trim13.States_(4).Known_ = [0; 1; 0]
  op_trim13.States_(4).Min_ = [0; -Inf; -Inf]
  op_trim13.States_(4).Max_ = [Inf; Inf; 0]
  op_trim13.Inputs_(1) = opcond.InputReport
  op_trim13.Inputs_(1).Block_ = 'trim1031/dE'
  op_trim13.Inputs_(1).PortWidth_ = 1
  op_trim13.Inputs_(1).PortDimensions_ = [1 1]
  op_trim13.Inputs_(1).u_ = -0.0124968353108
  op_trim13.Inputs_(1).Known_ = 0
  op_trim13.Inputs_(1).Min_ = -Inf
  op_trim13.Inputs_(1).Max_ = Inf
  op_trim13.Inputs_(2) = opcond.InputReport
  op_trim13.Inputs_(2).Block_ = 'trim1031/dT'
  op_trim13.Inputs_(2).PortWidth_ = 1
  op_trim13.Inputs_(2).PortDimensions_ = [1 1]
  op_trim13.Inputs_(2).u_ = 191999.999642
  op_trim13.Inputs_(2).Known_ = 0
  op_trim13.Inputs_(2).Min_ = -Inf
  op_trim13.Inputs_(2).Max_ = Inf
  op_trim13.Inputs_(3) = opcond.InputReport
  op_trim13.Inputs_(3).Block_ = 'trim1031/dA'
  op_trim13.Inputs_(3).PortWidth_ = 1
  op_trim13.Inputs_(3).PortDimensions_ = [1 1]
  op_trim13.Inputs_(3).u_ = -2.78444784735e-05
  op_trim13.Inputs_(3).Known_ = 0
  op_trim13.Inputs_(3).Min_ = -0.001
  op_trim13.Inputs_(3).Max_ = 0.001
  op_trim13.Inputs_(4) = opcond.InputReport
  op_trim13.Inputs_(4).Block_ = 'trim1031/dR'
  op_trim13.Inputs_(4).PortWidth_ = 1
  op_trim13.Inputs_(4).PortDimensions_ = [1 1]
  op_trim13.Inputs_(4).u_ = 0.00018916555193
  op_trim13.Inputs_(4).Known_ = 0
  op_trim13.Inputs_(4).Min_ = -0.001
  op_trim13.Inputs_(4).Max_ = 0.001
  op_trim14 = opcond.OperatingReport
  op_trim14.Outputs_ = opcond.OutputReport
  op_trim14.Outputs_.yspec_ = [0; 0; 0; 0; 0; 0; 0; 0; 0; 0; 0; 0]
  op_trim14.Outputs_.Block_ = 'trim1031/Output'
  op_trim14.Outputs_.PortWidth_ = 12
  op_trim14.Outputs_.PortNumber_ = NaN
  op_trim14.Outputs_.y_ = [0.0001; 0.117526200284; 6.28308530718; -0.000189020429197; 0.0101067920949; -2.02135516275e-05; 120.000004191; 0.0130344316639; 9.99959180984; 0; 0; -1500.0000002]
  op_trim14.Outputs_.Known_ = [0; 0; 0; 0; 0; 0; 0; 0; 0; 0; 0; 0]
  op_trim14.Outputs_.Min_ = [-Inf; -Inf; -Inf; -Inf; -Inf; -Inf; -Inf; -Inf; -Inf; -Inf; -Inf; -Inf]
  op_trim14.Outputs_.Max_ = [Inf; Inf; Inf; Inf; Inf; Inf; Inf; Inf; Inf; Inf; Inf; Inf]
  op_trim14.TerminationString_ = '成功满足工作点设定。'
  op_trim14.OptimizationOutput_.iterations = 3
  op_trim14.OptimizationOutput_.funcCount = 44
  op_trim14.OptimizationOutput_.lssteplength = 1
  op_trim14.OptimizationOutput_.stepsize = 6.32859168734e-11
  op_trim14.OptimizationOutput_.algorithm = 'active-set'
  op_trim14.OptimizationOutput_.firstorderopt = 0
  op_trim14.OptimizationOutput_.constrviolation = 7.22555348887e-11
  op_trim14.OptimizationOutput_.message = '找到满足约束的局部最小值。
    | 
    | 优化已完成，因为目标函数沿
    | 可行方向在最优性容差值范围内呈现非递减，
    | 并且在约束容差值范围内满足约束。
    | 
    | <停止条件详细信息>
    | 
    | 优化已完成: 一阶最优性测度 0.000000e+00 小于
    | options.OptimalityTolerance = 1.000000e-06，并且最大约束违反值
    | 7.225553e-11 小于 options.ConstraintTolerance = 1.000000e-06。'
  op_trim14.OptimizationOutput_.bestfeasible.x = [0.117526200284; -0.000189020429197; 0.0101067920949; -2.02135516275e-05; 120.000004191; 0.0130344316639; 9.99959180984; 0; -1500.0000002; -0.0749641146971; 192000; -2.93859951368e-05; 0.000201623113903]
  op_trim14.OptimizationOutput_.bestfeasible.fval = 0
  op_trim14.OptimizationOutput_.bestfeasible.constrviolation = 7.22555348887e-11
  op_trim14.OptimizationOutput_.bestfeasible.firstorderopt = 0
  op_trim14.OptimizationOutput_.progress = {'<font face="monospaced"; size=3><BR>', '正在优化以求解所有所需的 dx/dt=0、x(k+1)-x(k)=0 和 y=ydes。<BR>', ' <BR>', '(最大误差)模块<BR>', ' ---------------------------------------------------------<BR>', '(1.84926e-01) trim1031/B747 Dynamics动力学参数计算/6DOF Equations of Motion运动学/6DOF (Euler Angles)1/ub,vb,wb<BR>', '(1.49498e-03) trim1031/B747 Dynamics动力学参数计算/6DOF Equations of Motion运动学/6DOF (Euler Angles)1/Calculate DCM & Euler Angles/phi theta psi<BR>', '(7.22555e-11) trim1031/B747 Dynamics动力学参数计算/6DOF Equations of Motion运动学/6DOF (Euler Angles)1/Calculate DCM & Euler Angles/phi theta psi<BR>', '(7.22555e-11) trim1031/B747 Dynamics动力学参数计算/6DOF Equations of Motion运动学/6DOF (Euler Angles)1/Calculate DCM & Euler Angles/phi theta psi<BR>', ' <BR>', '成功满足工作点设定。<BR>'}
  op_trim14.Model_ = 'trim1031'
  op_trim14.States_(1) = opcond.StateReport
  op_trim14.States_(1).dx_ = [-0.000191287718347; 0.0101067940658; -1.93362588258e-05]
  op_trim14.States_(1).Nx_ = 3
  op_trim14.States_(1).Block_ = 'trim1031/B747 Dynamics动力学参数计算/6DOF Equations of Motion运动学/6DOF (Euler Angles)1/Calculate DCM &
    | Euler Angles/phi
    | theta
    | psi'
  op_trim14.States_(1).x_ = [0.0001; 0.117526200284; -0.0001]
  op_trim14.States_(1).SteadyState_ = [0; 0; 0]
  op_trim14.States_(1).dxMin_ = [-Inf; -0.2; -Inf]
  op_trim14.States_(1).dxMax_ = [Inf; 0.2; Inf]
  op_trim14.States_(1).Known_ = [1; 0; 1]
  op_trim14.States_(1).Min_ = [-Inf; -0.51; -Inf]
  op_trim14.States_(1).Max_ = [Inf; 0.51; Inf]
  op_trim14.States_(2) = opcond.StateReport
  op_trim14.States_(2).dx_ = [5.3121285559e-12; 2.4499302554e-12; 2.16996306049e-11]
  op_trim14.States_(2).Nx_ = 3
  op_trim14.States_(2).Block_ = 'trim1031/B747 Dynamics动力学参数计算/6DOF Equations of Motion运动学/6DOF (Euler Angles)1/p,q,r '
  op_trim14.States_(2).x_ = [-0.000189020429197; 0.0101067920949; -2.02135516275e-05]
  op_trim14.States_(2).SteadyState_ = [1; 1; 1]
  op_trim14.States_(2).dxMin_ = [-Inf; -0.02; -Inf]
  op_trim14.States_(2).dxMax_ = [Inf; 0.02; Inf]
  op_trim14.States_(2).Known_ = [0; 0; 0]
  op_trim14.States_(2).Min_ = [-Inf; -0.2; -Inf]
  op_trim14.States_(2).Max_ = [Inf; 0.2; Inf]
  op_trim14.States_(3) = opcond.StateReport
  op_trim14.States_(3).dx_ = [1.1026971003e-11; 1.5181931233e-12; -7.22555348887e-11]
  op_trim14.States_(3).Nx_ = 3
  op_trim14.States_(3).Block_ = 'trim1031/B747 Dynamics动力学参数计算/6DOF Equations of Motion运动学/6DOF (Euler Angles)1/ub,vb,wb'
  op_trim14.States_(3).x_ = [120.000004191; 0.0130344316639; 9.99959180984]
  op_trim14.States_(3).SteadyState_ = [1; 1; 1]
  op_trim14.States_(3).dxMin_ = [-Inf; -Inf; -Inf]
  op_trim14.States_(3).dxMax_ = [Inf; Inf; Inf]
  op_trim14.States_(3).Known_ = [0; 0; 0]
  op_trim14.States_(3).Min_ = [0; 0; 0]
  op_trim14.States_(3).Max_ = [Inf; Inf; Inf]
  op_trim14.States_(4) = opcond.StateReport
  op_trim14.States_(4).dx_ = [120.344724394; 7.5571276667e-14; -4.14008725619]
  op_trim14.States_(4).Nx_ = 3
  op_trim14.States_(4).Block_ = 'trim1031/B747 Dynamics动力学参数计算/6DOF Equations of Motion运动学/6DOF (Euler Angles)1/xe,ye,ze'
  op_trim14.States_(4).x_ = [0; 0; -1500.0000002]
  op_trim14.States_(4).SteadyState_ = [0; 1; 0]
  op_trim14.States_(4).dxMin_ = [-Inf; -Inf; -100]
  op_trim14.States_(4).dxMax_ = [Inf; Inf; 100]
  op_trim14.States_(4).Known_ = [0; 1; 0]
  op_trim14.States_(4).Min_ = [0; -Inf; -Inf]
  op_trim14.States_(4).Max_ = [Inf; Inf; 0]
  op_trim14.Inputs_(1) = opcond.InputReport
  op_trim14.Inputs_(1).Block_ = 'trim1031/dE'
  op_trim14.Inputs_(1).PortWidth_ = 1
  op_trim14.Inputs_(1).PortDimensions_ = [1 1]
  op_trim14.Inputs_(1).u_ = -0.0749641146971
  op_trim14.Inputs_(1).Known_ = 0
  op_trim14.Inputs_(1).Min_ = -Inf
  op_trim14.Inputs_(1).Max_ = Inf
  op_trim14.Inputs_(2) = opcond.InputReport
  op_trim14.Inputs_(2).Block_ = 'trim1031/dT'
  op_trim14.Inputs_(2).PortWidth_ = 1
  op_trim14.Inputs_(2).PortDimensions_ = [1 1]
  op_trim14.Inputs_(2).u_ = 192000
  op_trim14.Inputs_(2).Known_ = 0
  op_trim14.Inputs_(2).Min_ = -Inf
  op_trim14.Inputs_(2).Max_ = Inf
  op_trim14.Inputs_(3) = opcond.InputReport
  op_trim14.Inputs_(3).Block_ = 'trim1031/dA'
  op_trim14.Inputs_(3).PortWidth_ = 1
  op_trim14.Inputs_(3).PortDimensions_ = [1 1]
  op_trim14.Inputs_(3).u_ = -2.93859951368e-05
  op_trim14.Inputs_(3).Known_ = 0
  op_trim14.Inputs_(3).Min_ = -0.001
  op_trim14.Inputs_(3).Max_ = 0.001
  op_trim14.Inputs_(4) = opcond.InputReport
  op_trim14.Inputs_(4).Block_ = 'trim1031/dR'
  op_trim14.Inputs_(4).PortWidth_ = 1
  op_trim14.Inputs_(4).PortDimensions_ = [1 1]
  op_trim14.Inputs_(4).u_ = 0.000201623113903
  op_trim14.Inputs_(4).Known_ = 0
  op_trim14.Inputs_(4).Min_ = -0.001
  op_trim14.Inputs_(4).Max_ = 0.001
  op_trim15 : opcond.OperatingReport (value not decoded)
  op_trim16 : opcond.OperatingReport (value not decoded)
  op_trim17 : opcond.OperatingReport (value not decoded)
  op_trim2 : opcond.OperatingReport (value not decoded)
  op_trim20 : opcond.OperatingReport (value not decoded)
  op_trim21 : opcond.OperatingReport (value not decoded)
  op_trim22 : opcond.OperatingReport (value not decoded)
  op_trim23 : opcond.OperatingReport (value not decoded)
  op_trim24 : opcond.OperatingReport (value not decoded)
  op_trim25 : opcond.OperatingReport (value not decoded)
  op_trim28 : opcond.OperatingReport (value not decoded)
  op_trim29 : opcond.OperatingReport (value not decoded)
  op_trim3 : opcond.OperatingReport (value not decoded)
  op_trim30 : opcond.OperatingReport (value not decoded)
  op_trim31 : opcond.OperatingReport (value not decoded)
  op_trim32 : opcond.OperatingReport (value not decoded)
  op_trim33 : opcond.OperatingReport (value not decoded)
  op_trim34 : opcond.OperatingReport (value not decoded)
  op_trim35 : opcond.OperatingReport (value not decoded)
  op_trim37 : opcond.OperatingReport (value not decoded)
  op_trim39 : opcond.OperatingReport (value not decoded)
  op_trim4 : opcond.OperatingReport (value not decoded)
  op_trim42 : opcond.OperatingReport (value not decoded)
  op_trim45 : opcond.OperatingReport (value not decoded)
  op_trim48 : opcond.OperatingReport (value not decoded)
  op_trim49 : opcond.OperatingReport (value not decoded)
  op_trim5 : opcond.OperatingReport (value not decoded)
  op_trim6 : opcond.OperatingReport (value not decoded)
  op_trim69 : opcond.OperatingReport (value not decoded)
  op_trim7 : opcond.OperatingReport (value not decoded)
  op_trim8 : opcond.OperatingReport (value not decoded)
  op_trim9 : opcond.OperatingReport (value not decoded)
values from neighbouring files (symbols this model uses):
  B747 =     [B747.mat]
undefined symbols (not defined in the file or in its folder): Earth, env, WGS84
libraries: aerolibasang x2, sharedtransform x2, aerolibatmos2 x1, aerolibconvert2 x1, shared6dof x1, aerolibtransform2 x1
(part 1 of 2)
settings Model: Creator=Pro14  LastModifiedBy=阿汪
settings SolverCC: AlgebraicLoopSolver=TrustRegion
settings DataIOCC: ExternalInput=getinputstruct(op_trim29)  InitialState=getstatestruct(op_trim29)  LoadExternalInput=on  LoadInitialState=on
settings DebuggingCC: UnconnectedInputMsg=warning  UnconnectedOutputMsg=warning  UnconnectedLineMsg=warning
settings ModelReferenceCC: EnableRefExpFcnMdlSchedulingChecks=on
settings RTWCC: DLArmComputeVersion=19.05

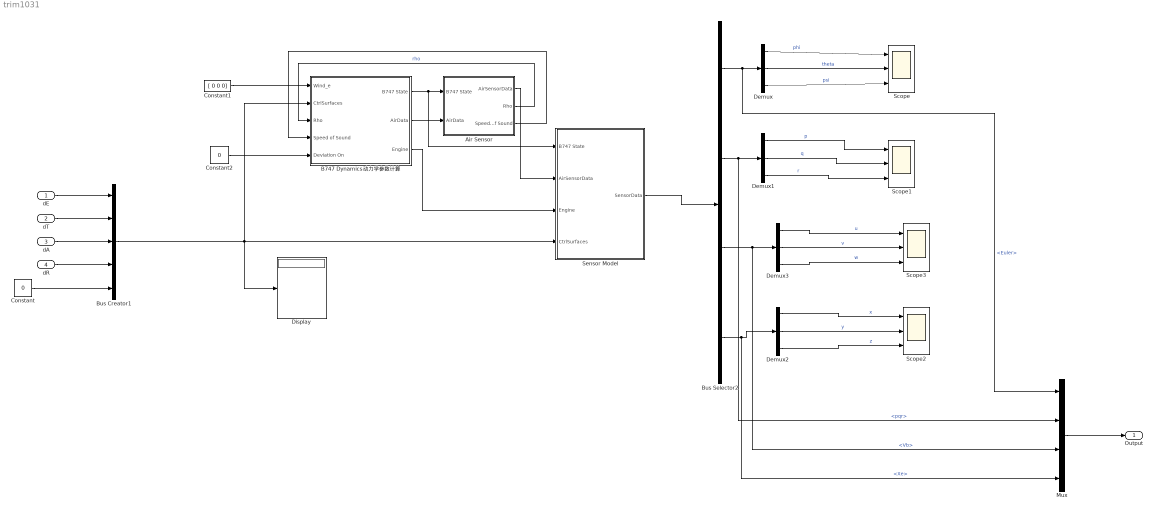
== system trim1031 ==
  dE : Inport
  dT : Inport  Port=2
  dA : Inport  Port=3
  dR : Inport  Port=4
  "Air Sensor " : Subsystem
  B747 Dynamics动力学参数计算 : Subsystem
  Bus Creator1 : BusCreator  Inputs=5
  Bus Selector2 : BusSelector  OutputSignals=Euler,pqr,Vb,Xe
  Constant : Constant  Value=0
  Constant1 : Constant  Value=[ 0 0 0]
      settings: AttributesFormatString=%<Value>
  Constant2 : Constant  Value=0
  Demux{,1..3} (4 alike) : Demux  Outputs=3
  Display : Display
  Mux : Mux
  Scope{,1..3} (4 alike) : Scope  NumInputPorts=3
  Sensor Model : Subsystem
  Output : Outport
  wires:
  dT/1 -> Bus Creator1/2
  dA/1 -> Bus Creator1/3
  "Air Sensor "/2(Rho) -> B747 Dynamics动力学参数计算/3(Rho)  "rho"
  Bus Selector2/4 -> Mux/4, Demux2/1  "<Xe>"
  B747 Dynamics动力学参数计算/3(Engine) -> Sensor Model/3(Engine)
  "Air Sensor "/1(AirSensorData) -> Sensor Model/2(AirSensorData)
  "Air Sensor "/3(Speed of Sound) -> B747 Dynamics动力学参数计算/4(Speed of Sound)
  B747 Dynamics动力学参数计算/2(AirData) -> "Air Sensor "/2(AirData)
  B747 Dynamics动力学参数计算/1(B747 State) -> Sensor Model/1(B747 State), "Air Sensor "/1(B747 State)
  dR/1 -> Bus Creator1/4
  Constant2/1 -> B747 Dynamics动力学参数计算/5(Deviation On)
  Sensor Model/1(SensorData) -> Bus Selector2/1
  Constant1/1 -> B747 Dynamics动力学参数计算/1(Wind_e)
  Bus Selector2/2 -> Mux/2, Demux1/1  "<pqr>"
  Bus Creator1/1 -> B747 Dynamics动力学参数计算/2(CtrlSurfaces), Display/1, Sensor Model/4(CtrlSurfaces)
  Bus Selector2/1 -> Mux/1, Demux/1  "<Euler>"
  Demux/1 -> Scope/1  "phi"
  Demux/2 -> Scope/2  "theta"
  Demux/3 -> Scope/3  "psi"
  Demux1/2 -> Scope1/2  "q"
  Demux1/3 -> Scope1/3  "r"
  Demux1/1 -> Scope1/1  "p"
  Demux2/2 -> Scope2/2  "y"
  Demux2/3 -> Scope2/3  "z"
  Demux2/1 -> Scope2/1  "x"
  Demux3/1 -> Scope3/1  "u"
  Demux3/2 -> Scope3/2  "v"
  Demux3/3 -> Scope3/3  "w"
  Bus Selector2/3 -> Mux/3, Demux3/1  "<Vb>"
  dE/1 -> Bus Creator1/1
  Constant/1 -> Bus Creator1/5
  Mux/1 -> Output/1

== system trim1031/Air Sensor  ==
  note: ias = V
  B747 State : Inport
  AirData : Inport  Port=2
  Bus Creator : BusCreator  Inputs=9
  Bus Selector1 : BusSelector  OutputSignals=airpseed,q,alpha,beta,Ma
  Bus Selector3 : BusSelector  OutputSignals=Xe
  Gain : Gain  Gain=-1
      settings: AttributesFormatString=Z to Alt
  Gain1 : Gain
  Get Z : Selector  InputPortWidth=3  IndexOptions=Index vector (dialog)  Indices=[3]  OutputSizes=[(-2)]
  ISA Atmosphere Model : aerolibatmos2/ISA Atmosphere Model  useExtended=off  action=Warning  custom=off  viscosityOut=off  g=9.80665  gamma=1.4  R=287.0531  L=0.0065  h_trop=11000  h_strat=20000  rho0=1.225  P0=101325  T0=288.15  h0=0
  Temperature Conversion : aerolibconvert2/Temperature Conversion  IU=K  OU=C
  AirSensorData : Outport
  Rho : Outport  Port=2
  Speed of Sound : Outport  Port=3
  wires:
  Bus Selector3/1 -> Get Z/1  "<Xe>"
  Temperature Conversion/1 -> Bus Creator/1  "OAT"
  Bus Selector1/1 -> Gain1/1, Bus Creator/4  "<airpseed>"
  Bus Selector1/2 -> Bus Creator/5  "<q>"
  ISA Atmosphere Model/1 -> Temperature Conversion/1  "OAT"
  Bus Creator/1 -> AirSensorData/1
  Gain/1 -> ISA Atmosphere Model/1
  ISA Atmosphere Model/3 -> Bus Creator/2  "static"
  ISA Atmosphere Model/2 -> Speed of Sound/1
  ISA Atmosphere Model/4 -> Bus Creator/3, Rho/1  "rho"
  AirData/1 -> Bus Selector1/1
  Get Z/1 -> Gain/1
  B747 State/1 -> Bus Selector3/1
  Bus Selector1/3 -> Bus Creator/6  "<alpha>"
  Bus Selector1/4 -> Bus Creator/7  "<beta>"
  Bus Selector1/5 -> Bus Creator/8  "<Ma>"
  Gain1/1 -> Bus Creator/9  "ias"

== system trim1031/B747 Dynamics动力学参数计算 ==
  note: 推力
  note: 速度、位置、欧拉角、pqr和加速度
  Wind_e : Inport
  CtrlSurfaces : Inport  Port=2
  Rho : Inport  Port=3
  Speed of Sound : Inport  Port=4
  Deviation On : Inport  Port=5
  6DOF Equations of Motion运动学 : Subsystem  VariantControl=use_aerospace_blocks == 1
  Forces and Moments动力学 : Subsystem
  B747 State : Outport
  AirData : Outport  Port=2
  Engine : Outport  Port=3
  wires:
  6DOF Equations of Motion运动学/1(B747 State) -> B747 State/1, Forces and Moments动力学/1(B747 State)
  CtrlSurfaces/1 -> Forces and Moments动力学/4(CtrlSurfaces)
  Rho/1 -> Forces and Moments动力学/3(Rho)
  Wind_e/1 -> Forces and Moments动力学/2(Wind_e)
  Forces and Moments动力学/1(AirData) -> AirData/1
  Forces and Moments动力学/2(FM_b) -> 6DOF Equations of Motion运动学/1(FM_b)
  Forces and Moments动力学/3(Engine) -> Engine/1
  Speed of Sound/1 -> Forces and Moments动力学/5(Speed of Sound)
  Deviation On/1 -> Forces and Moments动力学/6(Deviation On)
  Forces and Moments动力学/4(IsGround) -> 6DOF Equations of Motion运动学/2(IsGround)

== system trim1031/Sensor Model ==
  B747 State : Inport
  AirSensorData : Inport  Port=2
  Engine : Inport  Port=3
  CtrlSurfaces : Inport  Port=4
  Assemble GPS and State Data : Subsystem
  SensorData : Outport
  wires:
  AirSensorData/1 -> Assemble GPS and State Data/1(AirSensorData)
  CtrlSurfaces/1 -> Assemble GPS and State Data/3(CtrlSurfaces)
  B747 State/1 -> Assemble GPS and State Data/2(B747 State)
  Assemble GPS and State Data/1(B747 StateBus) -> SensorData/1  "B747 State"
  Engine/1 -> Assemble GPS and State Data/4(Engine)

== system trim1031/B747 Dynamics动力学参数计算/6DOF Equations of Motion运动学 ==
  FM_b : Inport
  IsGround : Inport  Port=2
  6DOF (Euler Angles)1 : shared6dof/6DOF (Euler Angles)  units=Metric (MKS)  mtype=Fixed  rep=Euler Angles  xme_0=B747.ic.Pos_0.*[1; 1; -1]  Vm_0=B747.ic.Vb_0  eul_0=B747.ic.Euler_0  pm_0=B747.ic.PQR_0  mass_0=B747.geometry.mass  mass_e=B747.geometry.massEmpty  mass_f=B747.geometry.massFull  inertia=diag([B747.inertia.Ixx B747.inertia.Iyy B747.inertia.Izz])  inertia_e=diag([B747.inertia.Ixx B747.inertia.Iyy B747.inertia.Izz])  inertia_f=diag([B747.inertia.Ixx B747.inertia.Iyy B747.inertia.Izz])  k_quat=1.0  vre_flag=off  abi_flag=off  aMode=aMode  xme_statename=''  Vm_statename=''  eul_statename=''  quat_statename=''  pm_statename=''  mass_statename=''
  Bus Creator : BusCreator  Inputs=8
  Compute psi_dot : Subsystem
  Demux2 : Demux  Outputs=2
  Terminator1 : Terminator
  Terminator2 : Terminator
  "[0, pi] Wrap Around" : Subsystem
  B747 State : Outport
  wires:
  6DOF (Euler Angles)1/8 -> Bus Creator/6  "Ab"
  "[0, pi] Wrap Around"/1(Wrapped) -> Bus Creator/3  "Euler"
  6DOF (Euler Angles)1/5 -> Bus Creator/4  "Vb"
  6DOF (Euler Angles)1/2 -> Bus Creator/2  "Xe"
  6DOF (Euler Angles)1/1 -> Bus Creator/1  "Ve"
  Bus Creator/1 -> B747 State/1
  6DOF (Euler Angles)1/4 -> Terminator1/1
  6DOF (Euler Angles)1/3 -> Compute psi_dot/1(Euler), "[0, pi] Wrap Around"/1(Euler)
  6DOF (Euler Angles)1/6 -> Compute psi_dot/2(G), Bus Creator/5  "pqr"
  FM_b/1 -> Demux2/1
  Demux2/1 -> 6DOF (Euler Angles)1/1
  Compute psi_dot/1(psi_dot) -> Bus Creator/7  "psi_dot"
  Demux2/2 -> 6DOF (Euler Angles)1/2
  6DOF (Euler Angles)1/7 -> Terminator2/1
  IsGround/1 -> Bus Creator/8  "IsGround"

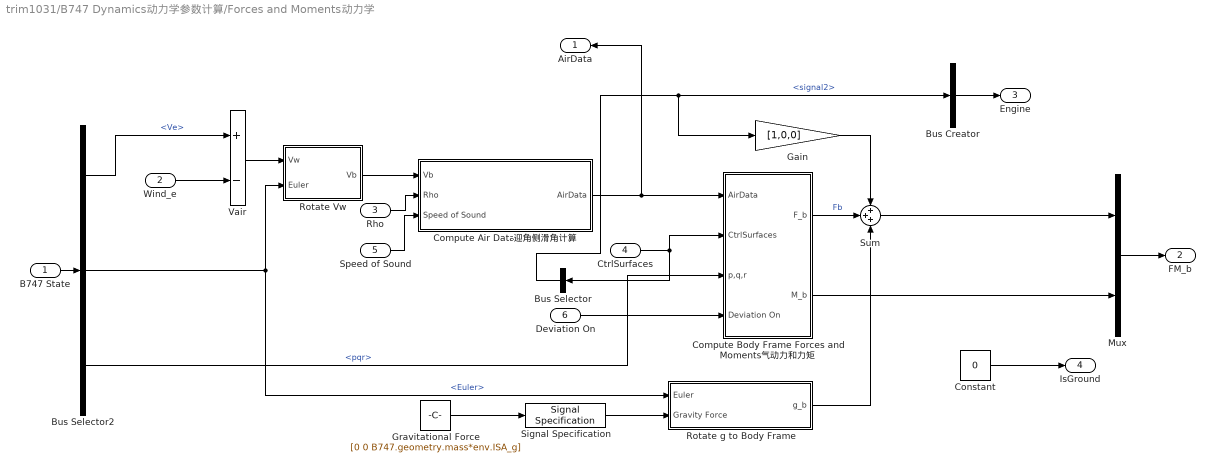
== system trim1031/B747 Dynamics动力学参数计算/Forces and Moments动力学 ==
  B747 State : Inport
  Wind_e : Inport  Port=2
  Rho : Inport  Port=3
  CtrlSurfaces : Inport  Port=4
  Speed of Sound : Inport  Port=5
  Deviation On : Inport  Port=6
  Bus Creator : BusCreator  Inputs=1
  Bus Selector : BusSelector  OutputSignals=signal2
  Bus Selector2 : BusSelector  OutputSignals=Ve,Euler,pqr
  Compute Air Data迎角侧滑角计算 : Subsystem  TreatAsAtomicUnit=on  VariantControl=use_aerospace_blocks == 1
  Compute Body Frame Forces and Moments气动力和力矩 : Subsystem
  Constant : Constant  Value=0
  Gain : Gain  Gain=[1,0,0]
  Gravitational Force : Constant  Value=[0 0 B747.geometry.mass*env.ISA_g]  VectorParams1D=off
      settings: AttributesFormatString=%<Value>
  Mux : Mux  Inputs=2
  Rotate Vw : Subsystem
  Rotate g to Body Frame : Subsystem
  Signal Specification : SignalSpecification
  Sum : Sum  Inputs=+++  SaturateOnIntegerOverflow=on
  Vair : Sum  Inputs=+-  InputSameDT=on  SaturateOnIntegerOverflow=on  OutDataTypeStr=Inherit: Same as first input
  AirData : Outport
  FM_b : Outport  Port=2
  Engine : Outport  Port=3
  IsGround : Outport  Port=4
  wires:
  Bus Selector2/1 -> Vair/1  "<Ve>"
  B747 State/1 -> Bus Selector2/1
  Mux/1 -> FM_b/1
  Compute Body Frame Forces and Moments气动力和力矩/1(F_b) -> Sum/2  "Fb"
  Rotate g to Body Frame/1(g_b) -> Sum/3
  Wind_e/1 -> Vair/2
  CtrlSurfaces/1 -> Compute Body Frame Forces and Moments气动力和力矩/2(CtrlSurfaces), Bus Selector/1
  Bus Selector2/3 -> Compute Body Frame Forces and Moments气动力和力矩/3(p,q,r)  "<pqr>"
  Gravitational Force/1 -> Signal Specification/1
  Rotate Vw/1(Vb) -> Compute Air Data迎角侧滑角计算/1(Vb)
  Rho/1 -> Compute Air Data迎角侧滑角计算/2(Rho)
  Bus Selector2/2 -> Rotate Vw/2(Euler), Rotate g to Body Frame/1(Euler)  "<Euler>"
  Vair/1 -> Rotate Vw/1(Vw)
  Signal Specification/1 -> Rotate g to Body Frame/2(Gravity Force)
  Sum/1 -> Mux/1
  Compute Body Frame Forces and Moments气动力和力矩/2(M_b) -> Mux/2
  Speed of Sound/1 -> Compute Air Data迎角侧滑角计算/3(Speed of Sound)
  Compute Air Data迎角侧滑角计算/1(AirData) -> AirData/1, Compute Body Frame Forces and Moments气动力和力矩/1(AirData)
  Bus Selector/1 -> Bus Creator/1, Gain/1  "<signal2>"
  Deviation On/1 -> Compute Body Frame Forces and Moments气动力和力矩/4(Deviation On)
  Bus Creator/1 -> Engine/1
  Constant/1 -> IsGround/1
  Gain/1 -> Sum/1

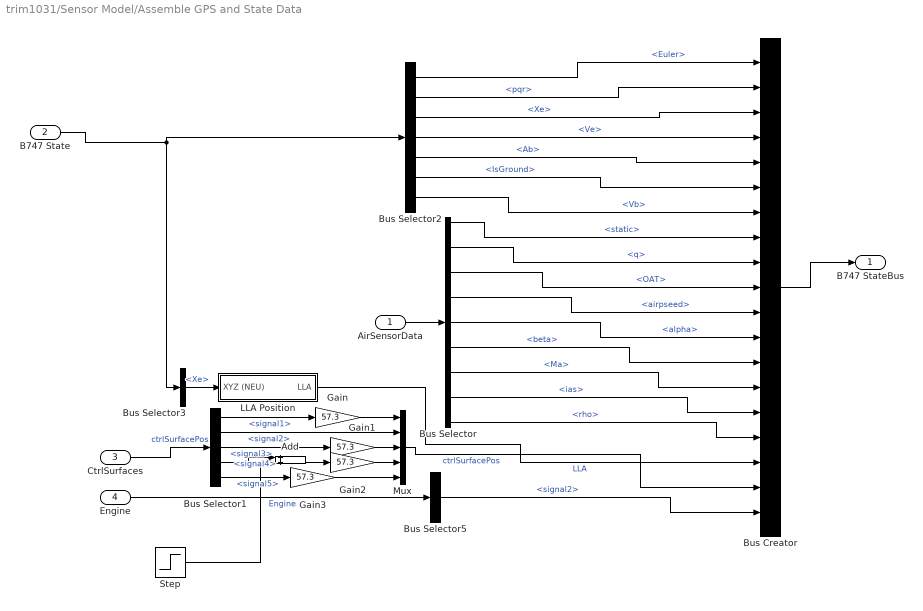
== system trim1031/Sensor Model/Assemble GPS and State Data ==
  AirSensorData : Inport
  B747 State : Inport  Port=2
  CtrlSurfaces : Inport  Port=3
  Engine : Inport  Port=4
  Add : Sum
  Bus Creator : BusCreator  Inputs=19
  Bus Selector : BusSelector  OutputSignals=static,q,OAT,airpseed,alpha,beta,Ma,ias,rho
  Bus Selector1 : BusSelector  OutputSignals=signal1,signal2,signal3,signal4,signal5
  Bus Selector2 : BusSelector  OutputSignals=Euler,pqr,Xe,Ve,Ab,IsGround,Vb
  Bus Selector3 : BusSelector  OutputSignals=Xe
  Bus Selector5 : BusSelector  OutputSignals=signal2
  Gain{,1..3} (4 alike) : Gain  Gain=57.3
  LLA Position : Subsystem
  Mux : Mux  Inputs=5
  Step : Step  Time=200  After=-0.0005  SampleTime=0
  B747 StateBus : Outport
  wires:
  Mux/1 -> Bus Creator/18  "ctrlSurfacePos"
  CtrlSurfaces/1 -> Bus Selector1/1  "ctrlSurfacePos"
  Bus Selector/4 -> Bus Creator/11  "<airpseed>"
  Bus Selector/3 -> Bus Creator/10  "<OAT>"
  Bus Selector/2 -> Bus Creator/9  "<q>"
  Bus Selector/1 -> Bus Creator/8  "<static>"
  Bus Selector2/5 -> Bus Creator/5  "<Ab>"
  Bus Selector2/4 -> Bus Creator/4  "<Ve>"
  Bus Selector2/2 -> Bus Creator/2  "<pqr>"
  Bus Selector2/1 -> Bus Creator/1  "<Euler>"
  Bus Creator/1 -> B747 StateBus/1
  B747 State/1 -> Bus Selector3/1, Bus Selector2/1
  Bus Selector3/1 -> LLA Position/1(XYZ (NEU))  "<Xe>"
  AirSensorData/1 -> Bus Selector/1
  Bus Selector2/3 -> Bus Creator/3  "<Xe>"
  Bus Selector/5 -> Bus Creator/12  "<alpha>"
  Bus Selector/6 -> Bus Creator/13  "<beta>"
  Engine/1 -> Bus Selector5/1  "Engine"
  Bus Selector5/1 -> Bus Creator/19  "<signal2>"
  Bus Selector/7 -> Bus Creator/14  "<Ma>"
  Bus Selector/8 -> Bus Creator/15  "<ias>"
  Bus Selector2/6 -> Bus Creator/6  "<IsGround>"
  LLA Position/1(LLA) -> Bus Creator/17  "LLA"
  Bus Selector1/1 -> Gain/1  "<signal1>"
  Bus Selector1/2 -> Mux/2  "<signal2>"
  Bus Selector1/3 -> Gain1/1  "<signal3>"
  Bus Selector1/4 -> Add/1  "<signal4>"
  Bus Selector1/5 -> Gain3/1  "<signal5>"
  Bus Selector/9 -> Bus Creator/16  "<rho>"
  Bus Selector2/7 -> Bus Creator/7  "<Vb>"
  Step/1 -> Add/2
  Add/1 -> Gain2/1
  Gain/1 -> Mux/1
  Gain1/1 -> Mux/3
  Gain2/1 -> Mux/4
  Gain3/1 -> Mux/5

== system trim1031/B747 Dynamics动力学参数计算/6DOF Equations of Motion运动学/Compute psi_dot ==
  Euler : Inport
  G : Inport  Port=2
  Mux1 : Mux  Inputs=2
  psidot : Fcn  Expr=(u[5]*sin(u[1])+u[6]*cos(u[1]))/cos(u[2])
  psi_dot : Outport
  wires:
  G/1 -> Mux1/2
  psidot/1 -> psi_dot/1  "psi_dot"
  Mux1/1 -> psidot/1
  Euler/1 -> Mux1/1

== system trim1031/B747 Dynamics动力学参数计算/6DOF Equations of Motion运动学/[0, pi] Wrap Around ==
  Euler : Inport
  Compare To Zero : Subsystem  mask(Compare To Zero){relop=>=, OutDataTypeStr=uint8, ZeroCross=off}
      mask prompts: relop "Simulink:masks:Operator_MP"; OutDataTypeStr "Simulink:masks:OutputDataType_MP"; ZeroCross "Simulink:masks:EnableZerocrossingDetection_MP"
      mask help: Simulink:masks:CompareToZero_MD
      mask init:
      | blkName = gcb;
      | 
      | if strcmp(get_param(gcbh,'OutDataTypeStr'),'boolean')
      | 	setValue = 'boolean';
      | else
      |     setValue = 'fixdt(0, 8)';
      | end
      | 
      | set_param([blkName,'/Compare'],'relop',relop, ...
      | 	'OutDataTypeStr', setValue, 'ZeroCross', ZeroCross);
      mask TypeOptions relop: == | ~= | < | <= | >= | >
      mask TypeOptions OutDataTypeStr: Simulink:masks:uint8 | Simulink:masks:boolean
      mask Callback ZeroCross: sl('zeroCrossEnable', gcbh);
      mask Display: disp([relop,' 0'])
  Logical Operator : Logic  Operator=NOT  AllPortsSameDT=off  OutDataTypeStr=boolean
  Merge : Merge  InitialOutput=0
  Mux2 : Mux  Inputs=2
  Negative Yaw : Subsystem
  Positive Yaw : Subsystem
  Selector1 : Selector  InputPortWidth=3  IndexOptions=Index vector (dialog)  Indices=[1 2]  OutputSizes=1
  Selector2 : Selector  InputPortWidth=3  IndexOptions=Index vector (dialog)  Indices=[3]  OutputSizes=1
  Wrapped : Outport
  wires:
  Negative Yaw/1(yaw_wr) -> Merge/2
  Positive Yaw/1(yaw_wr) -> Merge/1
  Merge/1 -> Mux2/2
  Logical Operator/1 -> Negative Yaw/Enable
  Compare To Zero/1(y) -> Logical Operator/1, Positive Yaw/Enable
  Selector2/1 -> Negative Yaw/1(yaw), Positive Yaw/1(yaw), Compare To Zero/1(u)
  Mux2/1 -> Wrapped/1
  Selector1/1 -> Mux2/1
  Euler/1 -> Selector1/1, Selector2/1

== system trim1031/B747 Dynamics动力学参数计算/Forces and Moments动力学/Compute Air Data迎角侧滑角计算 ==
  Vb : Inport  PortDimensions=3
  Rho : Inport  Port=2
  Speed of Sound : Inport  Port=3
  " " : aerolibasang/Incidence, Sideslip, & Airspeed
  Bus Creator : BusCreator  Inputs=5
  Dynamic Pressure动压 : Subsystem  mask(Dynamic Pressure){}
      mask help: aeroblks:aeroblkasang:blockDynamicPressureDesc
      mask init:
      | aeroicon('aeroblk');
      mask Help: eval('asbhelp');
      mask Display:
      | port_label('input',1,'V','texmode','on');
      | port_label('input',2,'\rho','texmode','on');
      | port_label('output',1,'q','texmode','on');
      | str = aeroimage('dynpres',gcb);
      | disp(str,'texmode','on');
  Mach Number : aerolibasang/Mach Number
  AirData : Outport
  wires:
  Bus Creator/1 -> AirData/1
  " "/1 -> Bus Creator/1  "alpha"
  Rho/1 -> Dynamic Pressure动压/2(Air Density)
  " "/3 -> Bus Creator/3  "airpseed"
  Dynamic Pressure动压/1(qbar) -> Bus Creator/4  "q"
  " "/2 -> Bus Creator/2  "beta"
  Mach Number/1 -> Bus Creator/5  "Ma"
  Vb/1 -> Mach Number/1, Dynamic Pressure动压/1(Velocity), " "/1
  Speed of Sound/1 -> Mach Number/2

== system trim1031/B747 Dynamics动力学参数计算/Forces and Moments动力学/Compute Body Frame Forces and Moments气动力和力矩 ==
  AirData : Inport
  CtrlSurfaces : Inport  Port=2
  p,q,r : Inport  Port=3
  Deviation On : Inport  Port=4
  Bus Selector : BusSelector  OutputSignals=alpha,beta
  Mux : Mux  Inputs=2
  Rotate FM to body frame : Subsystem
  Wind frame F& M 气动力计算 : Subsystem
  F_b : Outport
  M_b : Outport  Port=2
  wires:
  Mux/1 -> Rotate FM to body frame/2(alpha_beta)
  Bus Selector/2 -> Mux/2  "<beta>"
  Bus Selector/1 -> Mux/1  "<alpha>"
  Wind frame F& M 气动力计算/1(FM_w) -> Rotate FM to body frame/1(FM_w)  "FM_W"
  p,q,r/1 -> Wind frame F& M 气动力计算/3(p,q,r)
  Rotate FM to body frame/2(M_b) -> M_b/1
  Rotate FM to body frame/1(F_b) -> F_b/1
  CtrlSurfaces/1 -> Wind frame F& M 气动力计算/2(CtrlSurfaces)
  AirData/1 -> Bus Selector/1, Wind frame F& M 气动力计算/1(Airdata)
  Deviation On/1 -> Wind frame F& M 气动力计算/4(Deviation On)

== system trim1031/B747 Dynamics动力学参数计算/Forces and Moments动力学/Rotate Vw ==
  Vw : Inport
  Euler : Inport  Port=2
  RL2B : Subsystem
  RL2B * Vw : Product  Multiplication=Matrix(*)  InputSameDT=on  SaturateOnIntegerOverflow=on  OutDataTypeStr=Inherit: Same as first input
  Vb : Outport
  wires:
  RL2B * Vw/1 -> Vb/1
  Vw/1 -> RL2B * Vw/2
  RL2B/1(RL2B) -> RL2B * Vw/1
  Euler/1 -> RL2B/1(Euler)

== system trim1031/B747 Dynamics动力学参数计算/Forces and Moments动力学/Rotate g to Body Frame ==
  Euler : Inport
  Gravity Force : Inport  Port=2  PortDimensions=3
  Product1 : Product  Multiplication=Matrix(*)  InputSameDT=on  SaturateOnIntegerOverflow=on  OutDataTypeStr=Inherit: Same as first input
  RL2B : Subsystem
  g_b : Outport
  wires:
  Gravity Force/1 -> Product1/2
  Euler/1 -> RL2B/1(Euler)
  Product1/1 -> g_b/1
  RL2B/1(RL2B) -> Product1/1

== system trim1031/Sensor Model/Assemble GPS and State Data/LLA Position ==
  XYZ (NEU) : Inport
  Flat Earth to LLA1 : aerolibtransform2/Flat Earth to LLA  units=Metric (MKS)  ptype=Earth (WGS84)  F=1/298.257223563  R=6378137  refPosPort=off  LL0=B747.ic.gsLL  psi=0
  Mux : Mux  Inputs=2
  Zero level trust : Constant  Value=0
      settings: AttributesFormatString=%<Value>
  LLA : Outport
  wires:
  Flat Earth to LLA1/1 -> Mux/1  "gps_latLon"
  Zero level trust/1 -> Flat Earth to LLA1/2
  XYZ (NEU)/1 -> Flat Earth to LLA1/1
  Flat Earth to LLA1/2 -> Mux/2  "gps_h"
  Mux/1 -> LLA/1

== system trim1031/B747 Dynamics动力学参数计算/6DOF Equations of Motion运动学/[0, pi] Wrap Around/Compare To Zero ==
  u : Inport
  Compare : RelationalOperator  OutDataTypeStr=fixdt(0, 8)  ZeroCross=off
  Constant : Constant  DisableCoverage=on  Value=0  OutDataTypeStr=Inherit: Inherit via back propagation  PreserveConstantTs=on
  y : Outport
  wires:
  Constant/1 -> Compare/2
  u/1 -> Compare/1
  Compare/1 -> y/1

== system trim1031/B747 Dynamics动力学参数计算/6DOF Equations of Motion运动学/[0, pi] Wrap Around/Negative Yaw ==
  yaw : Inport
  Enable : EnablePort
  Abs : Abs  SaturateOnIntegerOverflow=off
  Constant1 : Constant  Value=2*pi
      settings: AttributesFormatString=%<Value>
  Constant2 : Constant  Value=2*pi
      settings: AttributesFormatString=%<Value>
  Math Function : Math  Operator=mod  SignedPower=on
  Sum : Sum  Inputs=|-+
  yaw_wr : Outport
  wires:
  Sum/1 -> yaw_wr/1
  Constant2/1 -> Sum/2
  Abs/1 -> Math Function/1
  Math Function/1 -> Sum/1
  Constant1/1 -> Math Function/2
  yaw/1 -> Abs/1

== system trim1031/B747 Dynamics动力学参数计算/6DOF Equations of Motion运动学/[0, pi] Wrap Around/Positive Yaw ==
  yaw : Inport
  Enable : EnablePort
  Constant1 : Constant  Value=2*pi
      settings: AttributesFormatString=%<Value>
  Math Function : Math  Operator=mod  SignedPower=on
  yaw_wr : Outport
  wires:
  Math Function/1 -> yaw_wr/1
  Constant1/1 -> Math Function/2
  yaw/1 -> Math Function/1

== system trim1031/B747 Dynamics动力学参数计算/Forces and Moments动力学/Compute Air Data迎角侧滑角计算/Dynamic Pressure动压 ==
  Velocity : Inport
  Air Density : Inport  Port=2
  1/2rhoV^2 : Gain  Gain=1/2  SaturateOnIntegerOverflow=on  OutDataTypeStr=Inherit: Same as input  ParamDataTypeStr=Inherit: Same as input
  Product2 : Product  InputSameDT=on  SaturateOnIntegerOverflow=on  OutDataTypeStr=Inherit: Same as first input
  dot : Subsystem
  qbar : Outport  InitialOutput=0
  wires:
  1/2rhoV^2/1 -> qbar/1
  Product2/1 -> 1/2rhoV^2/1
  Air Density/1 -> Product2/2
  dot/1(dot) -> Product2/1
  Velocity/1 -> dot/1(V)

== system trim1031/B747 Dynamics动力学参数计算/Forces and Moments动力学/Compute Body Frame Forces and Moments气动力和力矩/Rotate FM to body frame ==
  FM_w : Inport
  alpha_beta : Inport  Port=2
  Forces : Selector  InputPortWidth=6  IndexOptions=Index vector (dialog)  Indices=[1 2 3]  OutputSizes=[(-2)]
  Moments : Selector  InputPortWidth=6  IndexOptions=Index vector (dialog)  Indices=[4 5 6]  OutputSizes=[(-2)]
  Rotate Forces : Subsystem
  Rotate Moments : Subsystem
  F_b : Outport
  M_b : Outport  Port=2
  wires:
  alpha_beta/1 -> Rotate Forces/2(alpha_beta), Rotate Moments/1(alpha_beta)
  Moments/1 -> Rotate Moments/2(M_w)
  FM_w/1 -> Moments/1, Forces/1
  Forces/1 -> Rotate Forces/1(F_w)
  Rotate Moments/1(M_b) -> M_b/1
  Rotate Forces/1(F_b) -> F_b/1

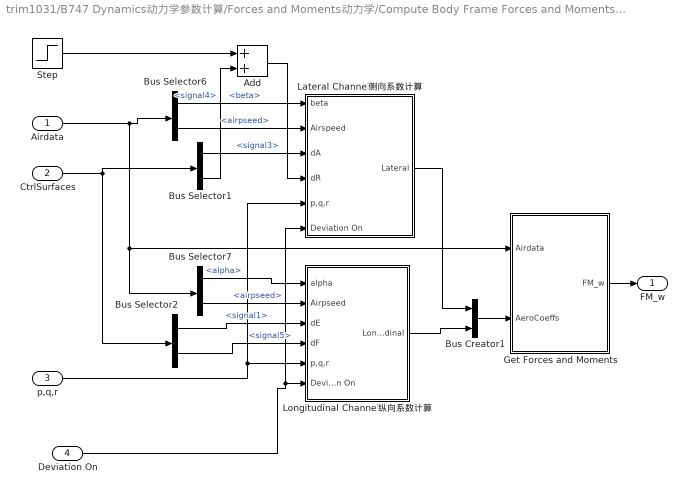
== system trim1031/B747 Dynamics动力学参数计算/Forces and Moments动力学/Compute Body Frame Forces and Moments气动力和力矩/Wind frame F& M 气动力计算 ==
  Airdata : Inport
  CtrlSurfaces : Inport  Port=2
  p,q,r : Inport  Port=3
  Deviation On : Inport  Port=4
  Add : Sum
  Bus Creator1 : BusCreator  Inputs=2
  Bus Selector1 : BusSelector  OutputSignals=signal3,signal4
  Bus Selector2 : BusSelector  OutputSignals=signal1,signal5
  Bus Selector6 : BusSelector  OutputSignals=beta,airpseed
  Bus Selector7 : BusSelector  OutputSignals=alpha,airpseed
  Get Forces and Moments : Subsystem
  Lateral Channel侧向系数计算 : Subsystem
  Longitudinal Channel纵向系数计算 : Subsystem
  Step : Step  Time=200  After=-0.0005  SampleTime=0
  FM_w : Outport  PortDimensions=6
  wires:
  Get Forces and Moments/1(FM_w) -> FM_w/1
  Bus Creator1/1 -> Get Forces and Moments/2(AeroCoeffs)
  Bus Selector7/2 -> Longitudinal Channel纵向系数计算/2(Airpseed)  "<airpseed>"
  Bus Selector7/1 -> Longitudinal Channel纵向系数计算/1(alpha)  "<alpha>"
  Bus Selector6/2 -> Lateral Channel侧向系数计算/2(Airspeed)  "<airpseed>"
  Bus Selector6/1 -> Lateral Channel侧向系数计算/1(beta)  "<beta>"
  Airdata/1 -> Bus Selector7/1, Get Forces and Moments/1(Airdata), Bus Selector6/1
  Bus Selector2/2 -> Longitudinal Channel纵向系数计算/4(dF)  "<signal5>"
  Bus Selector2/1 -> Longitudinal Channel纵向系数计算/3(dE)  "<signal1>"
  Bus Selector1/1 -> Lateral Channel侧向系数计算/3(dA)  "<signal3>"
  CtrlSurfaces/1 -> Bus Selector2/1, Bus Selector1/1
  p,q,r/1 -> Lateral Channel侧向系数计算/5(p,q,r), Longitudinal Channel纵向系数计算/5(p,q,r)
  Lateral Channel侧向系数计算/1(Lateral) -> Bus Creator1/1
  Longitudinal Channel纵向系数计算/1(Longitudinal) -> Bus Creator1/2
  Deviation On/1 -> Longitudinal Channel纵向系数计算/6(Deviation On), Lateral Channel侧向系数计算/6(Deviation On)
  Step/1 -> Add/1
  Bus Selector1/2 -> Add/2  "<signal4>"
  Add/1 -> Lateral Channel侧向系数计算/4(dR)

== system trim1031/B747 Dynamics动力学参数计算/Forces and Moments动力学/Rotate Vw/RL2B ==
  Euler : Inport
  Rotation Angles to Direction Cosine Matrix1 : sharedtransform/Rotation Angles to Direction Cosine Matrix  rotationOrder=ZYX  aMode=aMode
  Selector : Selector  InputPortWidth=3  IndexOptions=Index vector (dialog)  Indices=[3 2 1]  OutputSizes=1
  RL2B : Outport
  wires:
  Rotation Angles to Direction Cosine Matrix1/1 -> RL2B/1
  Euler/1 -> Selector/1
  Selector/1 -> Rotation Angles to Direction Cosine Matrix1/1

== system trim1031/B747 Dynamics动力学参数计算/Forces and Moments动力学/Rotate g to Body Frame/RL2B ==
  Euler : Inport
  Rotation Angles to Direction Cosine Matrix1 : sharedtransform/Rotation Angles to Direction Cosine Matrix  rotationOrder=ZYX  aMode=aMode
  Selector : Selector  InputPortWidth=3  IndexOptions=Index vector (dialog)  Indices=[3 2 1]  OutputSizes=1
  RL2B : Outport
  wires:
  Rotation Angles to Direction Cosine Matrix1/1 -> RL2B/1
  Euler/1 -> Selector/1
  Selector/1 -> Rotation Angles to Direction Cosine Matrix1/1

== system trim1031/B747 Dynamics动力学参数计算/Forces and Moments动力学/Compute Air Data迎角侧滑角计算/Dynamic Pressure动压/dot ==
  V : Inport
  Demux1 : Demux  Outputs=3
  Product : Product  RndMeth=Zero
  Product1 : Product  RndMeth=Zero
  Product2 : Product  RndMeth=Zero
  Sum : Sum  Inputs=+++
  dot : Outport
  wires:
  Product2/1 -> Sum/3
  Demux1/3 -> Product2/2, Product2/1
  Product/1 -> Sum/1
  Product1/1 -> Sum/2
  Sum/1 -> dot/1
  V/1 -> Demux1/1
  Demux1/1 -> Product/2, Product/1
  Demux1/2 -> Product1/1, Product1/2

== system trim1031/B747 Dynamics动力学参数计算/Forces and Moments动力学/Compute Body Frame Forces and Moments气动力和力矩/Rotate FM to body frame/Rotate Forces ==
  F_w : Inport
  alpha_beta : Inport  Port=2
  Math Function : Math  Operator=transpose  SignedPower=on
  Product2 : Product  Multiplication=Matrix(*)  SaturateOnIntegerOverflow=on  OutDataTypeStr=Inherit: Same as first input
  RB2W : Subsystem
  F_b : Outport  PortDimensions=3
  wires:
  F_w/1 -> Product2/2
  Product2/1 -> F_b/1
  alpha_beta/1 -> RB2W/1(aoa beta)
  Math Function/1 -> Product2/1
  RB2W/1(Rw2b) -> Math Function/1

== system trim1031/B747 Dynamics动力学参数计算/Forces and Moments动力学/Compute Body Frame Forces and Moments气动力和力矩/Rotate FM to body frame/Rotate Moments ==
  alpha_beta : Inport
  M_w : Inport  Port=2
  Math Function : Math  Operator=transpose  SignedPower=on
  Product2 : Product  Multiplication=Matrix(*)  SaturateOnIntegerOverflow=on  OutDataTypeStr=Inherit: Same as first input
  RB2W : Subsystem
  M_b : Outport  PortDimensions=3
  wires:
  RB2W/1(Rw2b) -> Math Function/1
  alpha_beta/1 -> RB2W/1(aoa beta)
  Product2/1 -> M_b/1
  M_w/1 -> Product2/2
  Math Function/1 -> Product2/1

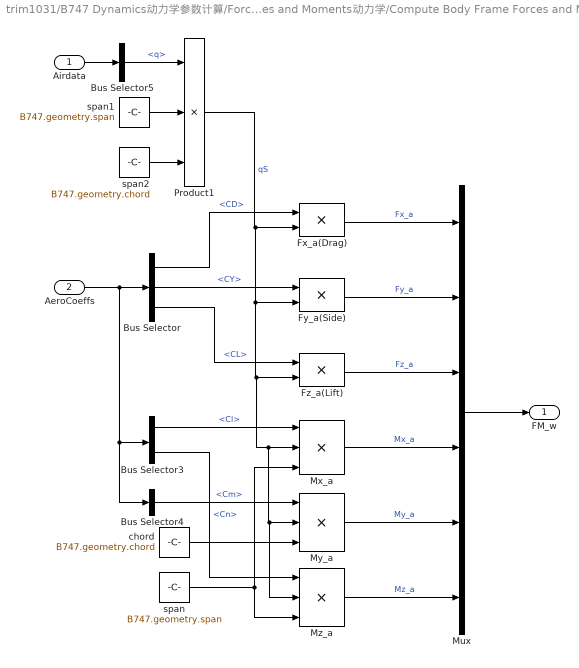
== system trim1031/B747 Dynamics动力学参数计算/Forces and Moments动力学/Compute Body Frame Forces and Moments气动力和力矩/Wind frame F& M 气动力计算/Get Forces and Moments ==
  Airdata : Inport
  AeroCoeffs : Inport  Port=2
  Bus Selector : BusSelector  OutputSignals=signal2.CD,signal1.CY,signal2.CL
  Bus Selector3 : BusSelector  OutputSignals=signal1.Cl,signal1.Cn
  Bus Selector4 : BusSelector  OutputSignals=signal2.Cm
  Bus Selector5 : BusSelector  OutputSignals=q
  Fx_a(Drag) : Product  Inputs=**  SaturateOnIntegerOverflow=on  OutDataTypeStr=Inherit: Same as first input
  Fy_a(Side) : Product  SaturateOnIntegerOverflow=on  OutDataTypeStr=Inherit: Same as first input
  Fz_a(Lift) : Product  SaturateOnIntegerOverflow=on  OutDataTypeStr=Inherit: Same as first input
  Mux : Mux  Inputs=6
  Mx_a : Product  Inputs=3  SaturateOnIntegerOverflow=on  OutDataTypeStr=Inherit: Same as first input
  My_a : Product  Inputs=3  SaturateOnIntegerOverflow=on  OutDataTypeStr=Inherit: Same as first input
  Mz_a : Product  Inputs=3  SaturateOnIntegerOverflow=on  OutDataTypeStr=Inherit: Same as first input
  Product1 : Product  Inputs=3  SaturateOnIntegerOverflow=on  OutDataTypeStr=Inherit: Same as first input
  chord : Constant  Value=B747.geometry.chord  VectorParams1D=off
      settings: AttributesFormatString=%<Value>
  span : Constant  Value=B747.geometry.span  VectorParams1D=off
      settings: AttributesFormatString=%<Value>
  span1 : Constant  Value=B747.geometry.span  VectorParams1D=off
      settings: AttributesFormatString=%<Value>
  span2 : Constant  Value=B747.geometry.chord  VectorParams1D=off
      settings: AttributesFormatString=%<Value>
  FM_w : Outport
  wires:
  Mx_a/1 -> Mux/4  "Mx_a"
  Bus Selector/2 -> Fy_a(Side)/1  "<CY>"
  Bus Selector4/1 -> My_a/1  "<Cm>"
  span2/1 -> Product1/3
  Fx_a(Drag)/1 -> Mux/1  "Fx_a"
  Bus Selector/1 -> Fx_a(Drag)/1  "<CD>"
  AeroCoeffs/1 -> Bus Selector/1, Bus Selector4/1, Bus Selector3/1
  My_a/1 -> Mux/5  "My_a"
  Fz_a(Lift)/1 -> Mux/3  "Fz_a"
  Mz_a/1 -> Mux/6  "Mz_a"
  Airdata/1 -> Bus Selector5/1
  chord/1 -> My_a/3
  span/1 -> Mz_a/3, Mx_a/3
  Fy_a(Side)/1 -> Mux/2  "Fy_a"
  Mux/1 -> FM_w/1
  Bus Selector3/2 -> Mz_a/1  "<Cn>"
  Bus Selector/3 -> Fz_a(Lift)/1  "<CL>"
  Product1/1 -> Fx_a(Drag)/2, Fy_a(Side)/2, Fz_a(Lift)/2, Mx_a/2, My_a/2, Mz_a/2  "qS"
  span1/1 -> Product1/2
  Bus Selector3/1 -> Mx_a/1  "<Cl>"
  Bus Selector5/1 -> Product1/1  "<q>"

== system trim1031/B747 Dynamics动力学参数计算/Forces and Moments动力学/Compute Body Frame Forces and Moments气动力和力矩/Wind frame F& M 气动力计算/Lateral Channel侧向系数计算 ==
  note: 偏航力矩系数
  note: 滚转力矩系数
  note: 侧力系数
  beta : Inport
  Airspeed : Inport  Port=2
  dA : Inport  Port=3
  dR : Inport  Port=4
  p,q,r : Inport  Port=5
  Deviation On : Inport  Port=6
  Bus Creator : BusCreator  Inputs=3
  CY : Subsystem
  Cl : Subsystem
  Cn : Subsystem
  Lateral : Outport
  wires:
  Cl/1(Cl) -> Bus Creator/2  "Cl"
  p,q,r/1 -> Cn/4(p,q,r), Cl/4(p,q,r)
  Airspeed/1 -> Cn/5(Airspeed), Cl/5(Airspeed)
  dR/1 -> CY/2(dR), Cl/3(dR), Cn/3(Dr)
  dA/1 -> Cn/2(dA), Cl/2(dA)
  beta/1 -> CY/1(beta), Cn/1(beta), Cl/1(beta)
  Cn/1(Cn) -> Bus Creator/3  "Cn"
  CY/1(CY) -> Bus Creator/1  "CY"
  Bus Creator/1 -> Lateral/1
  Deviation On/1 -> Cl/6(Deviation On)

== system trim1031/B747 Dynamics动力学参数计算/Forces and Moments动力学/Compute Body Frame Forces and Moments气动力和力矩/Wind frame F& M 气动力计算/Longitudinal Channel纵向系数计算 ==
  note: 俯仰力矩系数
  note: 升力系数
  note: 阻力系数
  alpha : Inport
  Airpseed : Inport  Port=2
  dE : Inport  Port=3
  dF : Inport  Port=4
  p,q,r : Inport  Port=5
  Deviation On : Inport  Port=6
  Bus Creator : BusCreator  Inputs=3
  CD : Subsystem
  CL : Subsystem
  Cm : Subsystem
  Y-down : Gain  Gain=-1  SaturateOnIntegerOverflow=on  OutDataTypeStr=Inherit: Same as input  ParamDataTypeStr=Inherit: Same as input
      settings: AttributesFormatString=%<Gain>
  Longitudinal : Outport
  wires:
  Airpseed/1 -> Cm/5(Airspeed), CL/6(Airspeed)
  p,q,r/1 -> Cm/4(p,q,r), CL/5(p,q,r)
  dF/1 -> Cm/3(Df), CL/4(dF)
  Bus Creator/1 -> Longitudinal/1
  Cm/1(Cm) -> Bus Creator/3  "Cm"
  CL/1(CL) -> Y-down/1
  dE/1 -> Cm/2(De), CL/3(dE)
  Y-down/1 -> Bus Creator/2  "CL"
  CD/1(CD) -> Bus Creator/1  "CD"
  alpha/1 -> CD/1(alpha), Cm/1(alpha), CL/2(alpha)
  Deviation On/1 -> Cm/6(Deviation On), CL/1(Deviation On), CD/2(Deviation On)

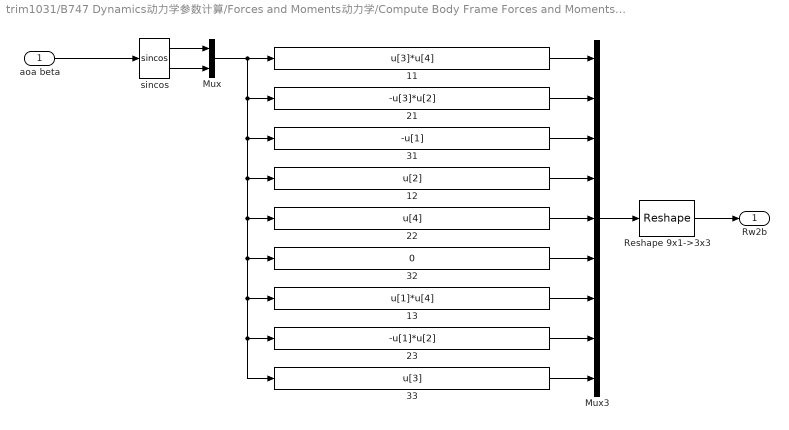
== system trim1031/B747 Dynamics动力学参数计算/Forces and Moments动力学/Compute Body Frame Forces and Moments气动力和力矩/Rotate FM to body frame/Rotate Forces/RB2W ==
  aoa beta : Inport
  11 : Fcn  Expr=u[3]*u[4]
  12 : Fcn  Expr=u[2]
  13 : Fcn  Expr=u[1]*u[4]
  21 : Fcn  Expr=-u[3]*u[2]
  22 : Fcn  Expr=u[4]
  23 : Fcn  Expr=-u[1]*u[2]
  31 : Fcn  Expr=-u[1]
  32 : Fcn  Expr=0
  33 : Fcn  Expr=u[3]
  Mux : Mux  Inputs=2
  Mux3 : Mux  Inputs=9
  Reshape 9x1->3x3 : Reshape  OutputDimensionality=Customize  OutputDimensions=[3,3]
  sincos : Trigonometry  Operator=sincos
  Rw2b : Outport
  wires:
  Mux/1 -> 11/1, 21/1, 31/1, 12/1, 22/1, 32/1, 13/1, 23/1, 33/1
  aoa beta/1 -> sincos/1
  sincos/2 -> Mux/2
  sincos/1 -> Mux/1
  33/1 -> Mux3/9
  23/1 -> Mux3/8
  13/1 -> Mux3/7
  32/1 -> Mux3/6
  22/1 -> Mux3/5
  12/1 -> Mux3/4
  31/1 -> Mux3/3
  21/1 -> Mux3/2
  11/1 -> Mux3/1
  Reshape 9x1->3x3/1 -> Rw2b/1
  Mux3/1 -> Reshape 9x1->3x3/1

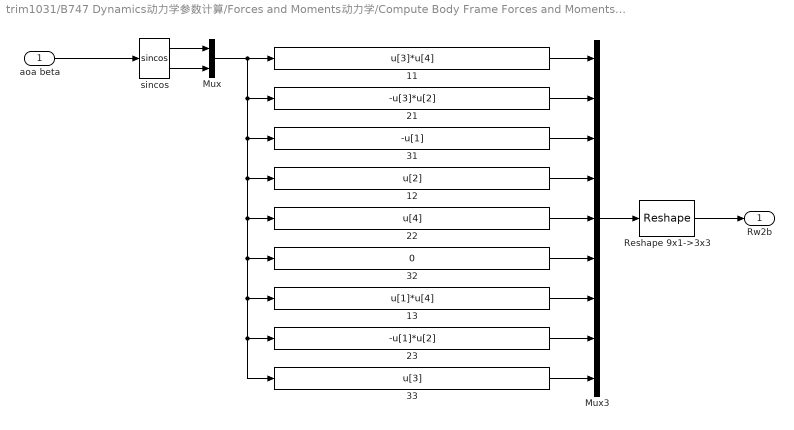
== system trim1031/B747 Dynamics动力学参数计算/Forces and Moments动力学/Compute Body Frame Forces and Moments气动力和力矩/Rotate FM to body frame/Rotate Moments/RB2W ==
  aoa beta : Inport
  11 : Fcn  Expr=u[3]*u[4]
  12 : Fcn  Expr=u[2]
  13 : Fcn  Expr=u[1]*u[4]
  21 : Fcn  Expr=-u[3]*u[2]
  22 : Fcn  Expr=u[4]
  23 : Fcn  Expr=-u[1]*u[2]
  31 : Fcn  Expr=-u[1]
  32 : Fcn  Expr=0
  33 : Fcn  Expr=u[3]
  Mux : Mux  Inputs=2
  Mux3 : Mux  Inputs=9
  Reshape 9x1->3x3 : Reshape  OutputDimensionality=Customize  OutputDimensions=[3,3]
  sincos : Trigonometry  Operator=sincos
  Rw2b : Outport
  wires:
  Mux/1 -> 11/1, 21/1, 31/1, 12/1, 22/1, 32/1, 13/1, 23/1, 33/1
  aoa beta/1 -> sincos/1
  sincos/2 -> Mux/2
  sincos/1 -> Mux/1
  33/1 -> Mux3/9
  23/1 -> Mux3/8
  13/1 -> Mux3/7
  32/1 -> Mux3/6
  22/1 -> Mux3/5
  12/1 -> Mux3/4
  31/1 -> Mux3/3
  21/1 -> Mux3/2
  11/1 -> Mux3/1
  Reshape 9x1->3x3/1 -> Rw2b/1
  Mux3/1 -> Reshape 9x1->3x3/1

== system trim1031/B747 Dynamics动力学参数计算/Forces and Moments动力学/Compute Body Frame Forces and Moments气动力和力矩/Wind frame F& M 气动力计算/Lateral Channel侧向系数计算/CY ==
  beta : Inport
  dR : Inport  Port=2
  CYDr : Constant  Value=B747.aero.CYDr
      settings: AttributesFormatString=%<Value>
  CYb : Constant  Value=B747.aero.CYb
      settings: AttributesFormatString=%<Value>
  Product : Product  SaturateOnIntegerOverflow=on  OutDataTypeStr=Inherit: Same as first input
  Product1 : Product  SaturateOnIntegerOverflow=on  OutDataTypeStr=Inherit: Same as first input
  Sum2 : Sum  SaturateOnIntegerOverflow=on
  CY : Outport
  wires:
  Product1/1 -> Sum2/2
  dR/1 -> Product1/2
  CYDr/1 -> Product1/1
  Product/1 -> Sum2/1
  Sum2/1 -> CY/1
  beta/1 -> Product/2
  CYb/1 -> Product/1

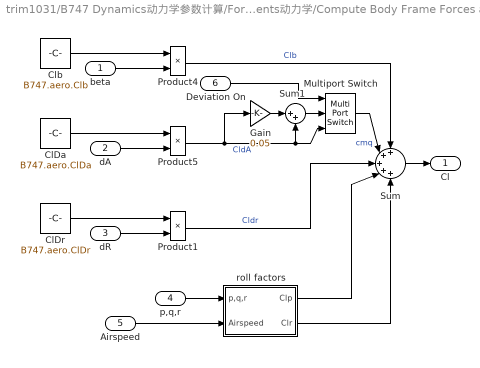
== system trim1031/B747 Dynamics动力学参数计算/Forces and Moments动力学/Compute Body Frame Forces and Moments气动力和力矩/Wind frame F& M 气动力计算/Lateral Channel侧向系数计算/Cl ==
  beta : Inport
  dA : Inport  Port=2
  dR : Inport  Port=3
  p,q,r : Inport  Port=4
  Airspeed : Inport  Port=5
  Deviation On : Inport  Port=6
  ClDa : Constant  Value=B747.aero.ClDa
      settings: AttributesFormatString=%<Value>
  ClDr : Constant  Value=B747.aero.ClDr
      settings: AttributesFormatString=%<Value>
  Clb : Constant  Value=B747.aero.Clb
      settings: AttributesFormatString=%<Value>
  Gain : Gain  Gain=0.05
  Multiport Switch : MultiPortSwitch  DataPortOrder=Specify indices  Inputs=2  DataPortIndices={1,0}  SaturateOnIntegerOverflow=off  InputSameDT=off
  Product1 : Product  SaturateOnIntegerOverflow=on  OutDataTypeStr=Inherit: Same as first input
  Product4 : Product  SaturateOnIntegerOverflow=on  OutDataTypeStr=Inherit: Same as first input
  Product5 : Product  SaturateOnIntegerOverflow=on  OutDataTypeStr=Inherit: Same as first input
  Sum : Sum  Inputs=+++++  SaturateOnIntegerOverflow=on
  Sum1 : Sum  Inputs=|++
  roll factors : Subsystem
  Cl : Outport
  wires:
  roll factors/1(Clp) -> Sum/4
  Product5/1 -> Gain/1, Sum1/2, Multiport Switch/3  "CldA"
  Airspeed/1 -> roll factors/2(Airspeed)
  p,q,r/1 -> roll factors/1(p,q,r)
  roll factors/2(Clr) -> Sum/5
  Product1/1 -> Sum/3  "Cldr"
  Product4/1 -> Sum/1  "Clb"
  Sum/1 -> Cl/1
  dR/1 -> Product1/2
  ClDr/1 -> Product1/1
  dA/1 -> Product5/2
  ClDa/1 -> Product5/1
  beta/1 -> Product4/2
  Clb/1 -> Product4/1
  Sum1/1 -> Multiport Switch/2
  Gain/1 -> Sum1/1
  Deviation On/1 -> Multiport Switch/1
  Multiport Switch/1 -> Sum/2  "cmq"

== system trim1031/B747 Dynamics动力学参数计算/Forces and Moments动力学/Compute Body Frame Forces and Moments气动力和力矩/Wind frame F& M 气动力计算/Lateral Channel侧向系数计算/Cn ==
  beta : Inport
  dA : Inport  Port=2
  Dr : Inport  Port=3
  p,q,r : Inport  Port=4
  Airspeed : Inport  Port=5
  CnDa : Constant  Value=B747.aero.CnDa
      settings: AttributesFormatString=%<Value>
  CnDr : Constant  Value=B747.aero.CnDr
      settings: AttributesFormatString=%<Value>
  Cnb : Constant  Value=B747.aero.Cnb
      settings: AttributesFormatString=%<Value>
  Product1 : Product  SaturateOnIntegerOverflow=on  OutDataTypeStr=Inherit: Same as first input
  Product4 : Product  SaturateOnIntegerOverflow=on  OutDataTypeStr=Inherit: Same as first input
  Product5 : Product  SaturateOnIntegerOverflow=on  OutDataTypeStr=Inherit: Same as first input
  Sum : Sum  Inputs=+++++  SaturateOnIntegerOverflow=on
  yaw factors : Subsystem
  Cn : Outport
  wires:
  Airspeed/1 -> yaw factors/2(Airspeed)
  p,q,r/1 -> yaw factors/1(p,q,r)
  Cnb/1 -> Product4/1
  beta/1 -> Product4/2
  CnDa/1 -> Product5/1
  Product5/1 -> Sum/2
  dA/1 -> Product5/2
  CnDr/1 -> Product1/1
  Dr/1 -> Product1/2
  Sum/1 -> Cn/1
  Product1/1 -> Sum/3
  yaw factors/2(Cnr) -> Sum/5
  yaw factors/1(Cnp) -> Sum/4
  Product4/1 -> Sum/1

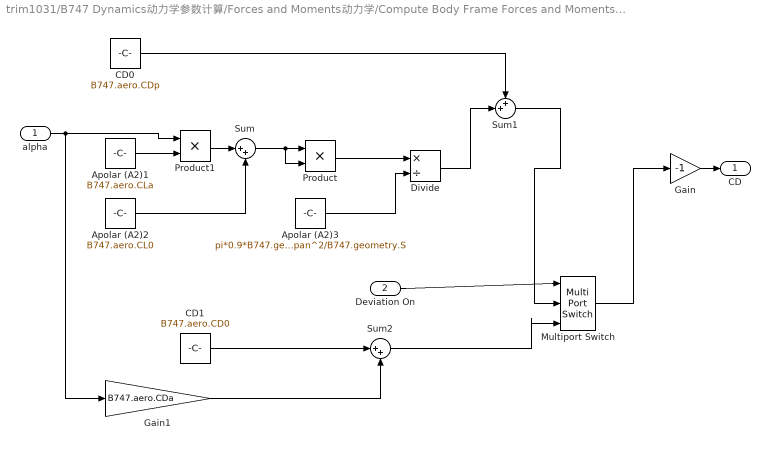
== system trim1031/B747 Dynamics动力学参数计算/Forces and Moments动力学/Compute Body Frame Forces and Moments气动力和力矩/Wind frame F& M 气动力计算/Longitudinal Channel纵向系数计算/CD ==
  alpha : Inport
  Deviation On : Inport  Port=2
  Apolar (A2)1 : Constant  Value=B747.aero.CLa
      settings: AttributesFormatString=%<Value>
  Apolar (A2)2 : Constant  Value=B747.aero.CL0
      settings: AttributesFormatString=%<Value>
  Apolar (A2)3 : Constant  Value=pi*0.9*B747.geometry.span^2/B747.geometry.S
      settings: AttributesFormatString=%<Value>
  CD0 : Constant  Value=B747.aero.CDp
      settings: AttributesFormatString=%<Value>
  CD1 : Constant  Value=B747.aero.CD0
      settings: AttributesFormatString=%<Value>
  Divide : Product  Inputs=*/
  Gain : Gain  Gain=-1  SaturateOnIntegerOverflow=on  OutDataTypeStr=Inherit: Same as input  ParamDataTypeStr=Inherit: Same as input
      settings: AttributesFormatString=%<Gain>
  Gain1 : Gain  Gain=B747.aero.CDa
  Multiport Switch : MultiPortSwitch  DataPortOrder=Specify indices  Inputs=2  DataPortIndices={1,0}  SaturateOnIntegerOverflow=off  InputSameDT=off
  Product : Product
  Product1 : Product
  Sum : Sum  Inputs=|++
  Sum1 : Sum  Inputs=++|  SaturateOnIntegerOverflow=on
  Sum2 : Sum  Inputs=|++
  CD : Outport
  wires:
  Gain/1 -> CD/1
  alpha/1 -> Gain1/1, Product1/1
  Sum1/1 -> Multiport Switch/2
  CD0/1 -> Sum1/1
  Apolar (A2)1/1 -> Product1/2
  Product1/1 -> Sum/1
  Apolar (A2)2/1 -> Sum/2
  Sum/1 -> Product/2, Product/1
  Product/1 -> Divide/1
  Apolar (A2)3/1 -> Divide/2
  Divide/1 -> Sum1/2
  CD1/1 -> Sum2/1
  Gain1/1 -> Sum2/2
  Sum2/1 -> Multiport Switch/3
  Deviation On/1 -> Multiport Switch/1
  Multiport Switch/1 -> Gain/1

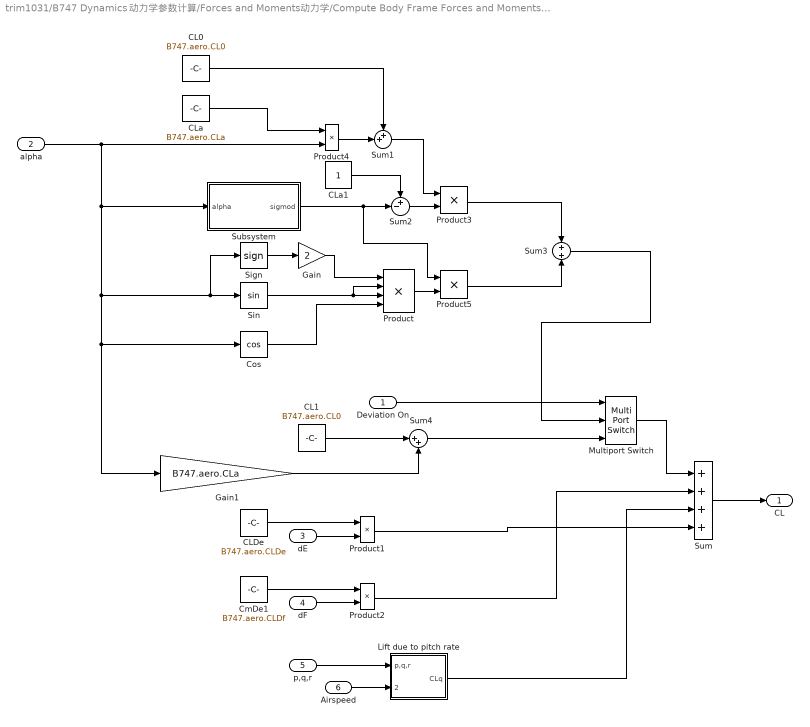
== system trim1031/B747 Dynamics动力学参数计算/Forces and Moments动力学/Compute Body Frame Forces and Moments气动力和力矩/Wind frame F& M 气动力计算/Longitudinal Channel纵向系数计算/CL ==
  Deviation On : Inport
  alpha : Inport  Port=2
  dE : Inport  Port=3
  dF : Inport  Port=4
  p,q,r : Inport  Port=5
  Airspeed : Inport  Port=6
  CL0 : Constant  Value=B747.aero.CL0
      settings: AttributesFormatString=%<Value>
  CL1 : Constant  Value=B747.aero.CL0
      settings: AttributesFormatString=%<Value>
  CLDe : Constant  Value=B747.aero.CLDe
      settings: AttributesFormatString=%<Value>
  CLa : Constant  Value=B747.aero.CLa
      settings: AttributesFormatString=%<Value>
  CLa1 : Constant
      settings: AttributesFormatString=%<Value>
  CmDe1 : Constant  Value=B747.aero.CLDf
      settings: AttributesFormatString=%<Value>
  Cos : Trigonometry  Operator=cos
  Gain : Gain  Gain=2
  Gain1 : Gain  Gain=B747.aero.CLa
  Lift due to pitch rate : Subsystem
  Multiport Switch : MultiPortSwitch  DataPortOrder=Specify indices  Inputs=2  DataPortIndices={1,0}  SaturateOnIntegerOverflow=off  InputSameDT=off
  Product : Product  Inputs=4
  Product1 : Product  SaturateOnIntegerOverflow=on  OutDataTypeStr=Inherit: Same as first input
  Product2 : Product  SaturateOnIntegerOverflow=on  OutDataTypeStr=Inherit: Same as first input
  Product3 : Product
  Product4 : Product  SaturateOnIntegerOverflow=on  OutDataTypeStr=Inherit: Same as first input
  Product5 : Product
  Sign : Signum
  Sin : Trigonometry
  Subsystem : Subsystem
  Sum : Sum  Inputs=++++  SaturateOnIntegerOverflow=on
  Sum1 : Sum  Inputs=++|
  Sum2 : Sum  Inputs=+-|
  Sum3 : Sum
  Sum4 : Sum  Inputs=|++
  CL : Outport
  wires:
  Airspeed/1 -> Lift due to pitch rate/2(Airspeed)
  p,q,r/1 -> Lift due to pitch rate/1(p,q,r)
  Lift due to pitch rate/1(CLq) -> Sum/3
  Product2/1 -> Sum/2
  Product1/1 -> Sum/4
  CmDe1/1 -> Product2/1
  dF/1 -> Product2/2
  Sum/1 -> CL/1
  dE/1 -> Product1/2
  CLDe/1 -> Product1/1
  alpha/1 -> Gain1/1, Cos/1, Sign/1, Sin/1, Subsystem/1(alpha), Product4/2
  CLa/1 -> Product4/1
  Product4/1 -> Sum1/2
  CL0/1 -> Sum1/1
  Sin/1 -> Product/3, Product/2
  Sign/1 -> Gain/1
  Gain/1 -> Product/1
  Cos/1 -> Product/4
  CLa1/1 -> Sum2/1
  Subsystem/1(sigmod) -> Product5/1, Sum2/2
  Sum2/1 -> Product3/2
  Sum1/1 -> Product3/1
  Product/1 -> Product5/2
  Product5/1 -> Sum3/2
  Product3/1 -> Sum3/1
  Sum3/1 -> Multiport Switch/2
  Multiport Switch/1 -> Sum/1
  CL1/1 -> Sum4/1
  Gain1/1 -> Sum4/2
  Sum4/1 -> Multiport Switch/3
  Deviation On/1 -> Multiport Switch/1

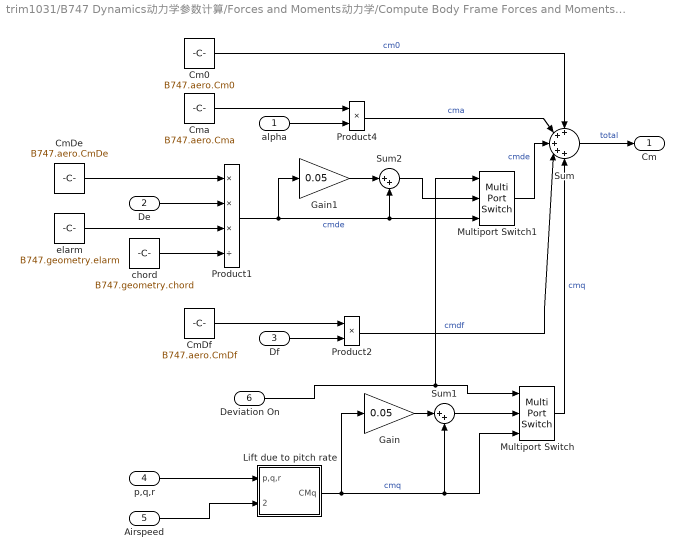
== system trim1031/B747 Dynamics动力学参数计算/Forces and Moments动力学/Compute Body Frame Forces and Moments气动力和力矩/Wind frame F& M 气动力计算/Longitudinal Channel纵向系数计算/Cm ==
  alpha : Inport
  De : Inport  Port=2
  Df : Inport  Port=3
  p,q,r : Inport  Port=4
  Airspeed : Inport  Port=5
  Deviation On : Inport  Port=6
  Cm0 : Constant  Value=B747.aero.Cm0
      settings: AttributesFormatString=%<Value>
  CmDe : Constant  Value=B747.aero.CmDe
      settings: AttributesFormatString=%<Value>
  CmDf : Constant  Value=B747.aero.CmDf
      settings: AttributesFormatString=%<Value>
  Cma : Constant  Value=B747.aero.Cma
      settings: AttributesFormatString=%<Value>
  Gain : Gain  Gain=0.05
  Gain1 : Gain  Gain=0.05
  Lift due to pitch rate : Subsystem
  Multiport Switch : MultiPortSwitch  DataPortOrder=Specify indices  Inputs=2  DataPortIndices={1,0}  SaturateOnIntegerOverflow=off  InputSameDT=off
  Multiport Switch1 : MultiPortSwitch  DataPortOrder=Specify indices  Inputs=2  DataPortIndices={1,0}  SaturateOnIntegerOverflow=off  InputSameDT=off
  Product1 : Product  Inputs=***/  SaturateOnIntegerOverflow=on  OutDataTypeStr=Inherit: Same as first input
  Product2 : Product  SaturateOnIntegerOverflow=on  OutDataTypeStr=Inherit: Same as first input
  Product4 : Product  SaturateOnIntegerOverflow=on  OutDataTypeStr=Inherit: Same as first input
  Sum : Sum  Inputs=+++++  SaturateOnIntegerOverflow=on
  Sum1 : Sum  Inputs=|++
  Sum2 : Sum  Inputs=|++
  chord : Constant  Value=B747.geometry.chord
      settings: AttributesFormatString=%<Value>
  elarm : Constant  Value=B747.geometry.elarm
      settings: AttributesFormatString=%<Value>
  Cm : Outport
  wires:
  chord/1 -> Product1/4
  elarm/1 -> Product1/3
  Multiport Switch/1 -> Sum/5  "cmq"
  p,q,r/1 -> Lift due to pitch rate/1(p,q,r)
  Multiport Switch1/1 -> Sum/3  "cmde"
  Product4/1 -> Sum/2  "cma"
  Sum/1 -> Cm/1  "total"
  De/1 -> Product1/2
  CmDe/1 -> Product1/1
  alpha/1 -> Product4/2
  Cma/1 -> Product4/1
  Df/1 -> Product2/2
  CmDf/1 -> Product2/1
  Product2/1 -> Sum/4  "cmdf"
  Cm0/1 -> Sum/1  "cm0"
  Airspeed/1 -> Lift due to pitch rate/2(Airspeed)
  Lift due to pitch rate/1(CMq) -> Gain/1, Sum1/2, Multiport Switch/3  "cmq"
  Gain/1 -> Sum1/1
  Sum1/1 -> Multiport Switch/2
  Deviation On/1 -> Multiport Switch1/1, Multiport Switch/1
  Product1/1 -> Gain1/1, Sum2/2, Multiport Switch1/3  "cmde"
  Gain1/1 -> Sum2/1
  Sum2/1 -> Multiport Switch1/2

== system trim1031/B747 Dynamics动力学参数计算/Forces and Moments动力学/Compute Body Frame Forces and Moments气动力和力矩/Wind frame F& M 气动力计算/Lateral Channel侧向系数计算/Cl/roll factors ==
  p,q,r : Inport
  Airspeed : Inport  Port=2
  Constant : Constant  Value=B747.aero.Clp
      settings: AttributesFormatString=%<Value>
  Constant1 : Constant  Value=B747.aero.Clr
      settings: AttributesFormatString=%<Value>
  Get p : Selector  InputPortWidth=3  IndexOptions=Index vector (dialog)  Indices=1  OutputSizes=[(-2)]
  Get r : Selector  InputPortWidth=3  IndexOptions=Index vector (dialog)  Indices=3  OutputSizes=[(-2)]
  Product : Product  SaturateOnIntegerOverflow=on  OutDataTypeStr=Inherit: Same as first input
  Product1 : Product  SaturateOnIntegerOverflow=on  OutDataTypeStr=Inherit: Same as first input
  roll rate fact : Subsystem
  yaw rate fact : Subsystem
  Clp : Outport
  Clr : Outport  Port=2
  wires:
  Get r/1 -> yaw rate fact/1(r)
  p,q,r/1 -> Get r/1, Get p/1
  Get p/1 -> roll rate fact/1(p)
  Airspeed/1 -> yaw rate fact/2(Airspeed), roll rate fact/2(Airspeed)
  yaw rate fact/1(Yaw Rate Fac) -> Product1/2
  Constant1/1 -> Product1/1
  roll rate fact/1(Roll Rate Fac) -> Product/2
  Constant/1 -> Product/1
  Product1/1 -> Clr/1
  Product/1 -> Clp/1

== system trim1031/B747 Dynamics动力学参数计算/Forces and Moments动力学/Compute Body Frame Forces and Moments气动力和力矩/Wind frame F& M 气动力计算/Lateral Channel侧向系数计算/Cn/yaw factors ==
  p,q,r : Inport
  Airspeed : Inport  Port=2
  Constant : Constant  Value=B747.aero.Cnp
      settings: AttributesFormatString=%<Value>
  Constant1 : Constant  Value=B747.aero.Cnr
      settings: AttributesFormatString=%<Value>
  Get p : Selector  InputPortWidth=3  IndexOptions=Index vector (dialog)  Indices=1  OutputSizes=[(-2)]
  Get r : Selector  InputPortWidth=3  IndexOptions=Index vector (dialog)  Indices=3  OutputSizes=[(-2)]
  Product : Product  SaturateOnIntegerOverflow=on  OutDataTypeStr=Inherit: Same as first input
  Product1 : Product  SaturateOnIntegerOverflow=on  OutDataTypeStr=Inherit: Same as first input
  roll rate fact : Subsystem
  yaw rate fact : Subsystem
  Cnp : Outport
  Cnr : Outport  Port=2
  wires:
  Airspeed/1 -> yaw rate fact/2(Airspeed), roll rate fact/2(Airspeed)
  Get r/1 -> yaw rate fact/1(r)
  p,q,r/1 -> Get r/1, Get p/1
  Get p/1 -> roll rate fact/1(p)
  roll rate fact/1(Roll Rate Fac) -> Product/2
  Constant/1 -> Product/1
  yaw rate fact/1(Yaw Rate Fac) -> Product1/2
  Constant1/1 -> Product1/1
  Product1/1 -> Cnr/1
  Product/1 -> Cnp/1

== system trim1031/B747 Dynamics动力学参数计算/Forces and Moments动力学/Compute Body Frame Forces and Moments气动力和力矩/Wind frame F& M 气动力计算/Longitudinal Channel纵向系数计算/CL/Lift due to pitch rate ==
  p,q,r : Inport
  Airspeed : Inport  Port=2
  Constant : Constant  Value=B747.aero.CLq
      settings: AttributesFormatString=%<Value>
  Get q : Selector  InputPortWidth=3  IndexOptions=Index vector (dialog)  Indices=2  OutputSizes=[(-2)]
  Product : Product  SaturateOnIntegerOverflow=on  OutDataTypeStr=Inherit: Same as first input
  pitch rate factor : Subsystem
  CLq : Outport
  wires:
  Airspeed/1 -> pitch rate factor/2(Airspeed)
  Get q/1 -> pitch rate factor/1(q)
  p,q,r/1 -> Get q/1
  Product/1 -> CLq/1
  pitch rate factor/1(Pitch Rate Fac) -> Product/2
  Constant/1 -> Product/1

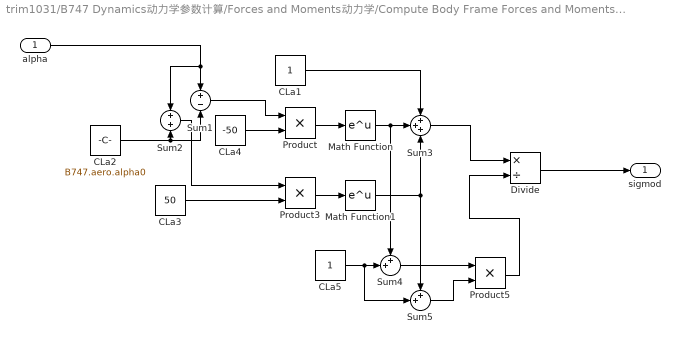
== system trim1031/B747 Dynamics动力学参数计算/Forces and Moments动力学/Compute Body Frame Forces and Moments气动力和力矩/Wind frame F& M 气动力计算/Longitudinal Channel纵向系数计算/CL/Subsystem ==
  alpha : Inport
  CLa1 : Constant
      settings: AttributesFormatString=%<Value>
  CLa2 : Constant  Value=B747.aero.alpha0
      settings: AttributesFormatString=%<Value>
  CLa3 : Constant  Value=50
      settings: AttributesFormatString=%<Value>
  CLa4 : Constant  Value=-50
      settings: AttributesFormatString=%<Value>
  CLa5 : Constant
      settings: AttributesFormatString=%<Value>
  Divide : Product  Inputs=*/
  Math Function : Math  SignedPower=on
  Math Function1 : Math  SignedPower=on
  Product : Product
  Product3 : Product
  Product5 : Product
  Sum1 : Sum  Inputs=+-
  Sum2 : Sum
  Sum3 : Sum  Inputs=+++
  Sum4 : Sum  Inputs=++|
  Sum5 : Sum  Inputs=++|
  sigmod : Outport
  wires:
  CLa5/1 -> Sum5/2, Sum4/2
  Sum4/1 -> Product5/1
  Sum5/1 -> Product5/2
  Math Function/1 -> Sum3/2, Sum4/1
  Sum3/1 -> Divide/1
  Product5/1 -> Divide/2
  CLa2/1 -> Sum1/2, Sum2/2
  CLa4/1 -> Product/2
  CLa1/1 -> Sum3/1
  Product/1 -> Math Function/1
  Sum1/1 -> Product/1
  Sum2/1 -> Product3/1
  Math Function1/1 -> Sum3/3, Sum5/1
  Product3/1 -> Math Function1/1
  CLa3/1 -> Product3/2
  Divide/1 -> sigmod/1
  alpha/1 -> Sum2/1, Sum1/1

== system trim1031/B747 Dynamics动力学参数计算/Forces and Moments动力学/Compute Body Frame Forces and Moments气动力和力矩/Wind frame F& M 气动力计算/Longitudinal Channel纵向系数计算/Cm/Lift due to pitch rate ==
  p,q,r : Inport
  Airspeed : Inport  Port=2
  Cma1 : Constant  Value=B747.aero.Cmq
      settings: AttributesFormatString=%<Value>
  Get q : Selector  InputPortWidth=3  IndexOptions=Index vector (dialog)  Indices=2  OutputSizes=[(-2)]
  Product : Product  SaturateOnIntegerOverflow=on  OutDataTypeStr=Inherit: Same as first input
  pitch rate factor : Subsystem
  CMq : Outport
  wires:
  Airspeed/1 -> pitch rate factor/2(Airspeed)
  Get q/1 -> pitch rate factor/1(q)
  p,q,r/1 -> Get q/1
  Product/1 -> CMq/1
  pitch rate factor/1(Pitch Rate Fac) -> Product/2
  Cma1/1 -> Product/1
